simulink model "solution1_7009_CAN"  (R2017b)
settings: Solver=FixedStepAuto  StartTime=0.0  StopTime=inf  FixedStep=0.01  RelTol=1e-3
PostLoadFcn:
  | , if any(exist('dsrtsu_mdlpostloadfcn', 'file') == [2, 3, 6]), try dsrtsu_mdlpostloadfcn('Execute', bdroot); catch fprintf('Error in PostLoadFcn (dsrtsu_mdlpostloadfcn) for model "%s":\n %s\n', bdroot, lasterr); end, end,
values from neighbouring files (symbols this model uses):
  g = 9.81    [initialize_simplemodel.m]    (also in initialize_simplemodel_Trial.m; tire_friction_circle.m)
  h = 0.35    [initialize_simplemodel.m]    (also in initialize_simplemodel_Trial.m)
  lf = 1.4    [initialize_simplemodel.m]    (also in initialize_simplemodel_Trial.m)
  lr = 1.345    [initialize_simplemodel.m]    (also in initialize_simplemodel_Trial.m)
  m = 1400    [initialize_simplemodel.m]    (also in initialize_simplemodel_Trial.m = 1300; tire_friction_circle.m = 1300)
  r = 0.34    [initialize_simplemodel.m]    (also in initialize_simplemodel_Trial.m)
  tr = 1.684/2    (= 0.842)    [initialize_simplemodel.m]    (also in initialize_simplemodel_Trial.m)
  v_init = 60*5/18    (= 16.6666666667)    [initialize_simplemodel.m]    (also in initialize_simplemodel_Trial.m)
undefined symbols (not defined in the file or in its folder): DiscIntNeverNeededParam
libraries: simulink x27, rtican x10
(part 1 of 3)
settings Model: DSRTSU_INTERNAL_RTI_VER=510  DSRTSU_INTERNAL_RTI_TYPE=rti1401  Creator=ashwin.ramanujam  LastModifiedBy=Dell
settings DataIOCC: SignalLogging=off
settings HardwareCC: ProdBitPerPointer=32  ProdBitPerSizeT=32  ProdBitPerPtrDiffT=32  ProdLargestAtomicInteger=Integer  ProdEndianess=BigEndian  ProdWordSize=32  ProdHWDeviceType=Custom Processor->Custom  TargetIntDivRoundTo=Zero  TargetEndianess=BigEndian  TargetHWDeviceType=Custom Processor->Custom
settings SFSimCC: MATLABDynamicMemAlloc=off
settings RTWCC: SystemTargetFile=rti1401.tlc  MakeCommand=make_rti  TemplateMakefile=rti1401.tmf  Description=dSPACE DS1401 Hardware Platform
settings STFCustomTargetCC: ParMdlRefBuildCompliant=on  GRTInterface=off  SystemTargetFile=rti1401.tlc
settings GRTTargetCC: TargetLangStandard=C89/C90 (ANSI)  CompOptLevelCompliant=off  ConcurrentExecutionCompliant=off  CombineOutputUpdateFcns=off  MatFileLogging=off  CPPClassGenCompliant=off  UseToolchainInfoCompliant=off

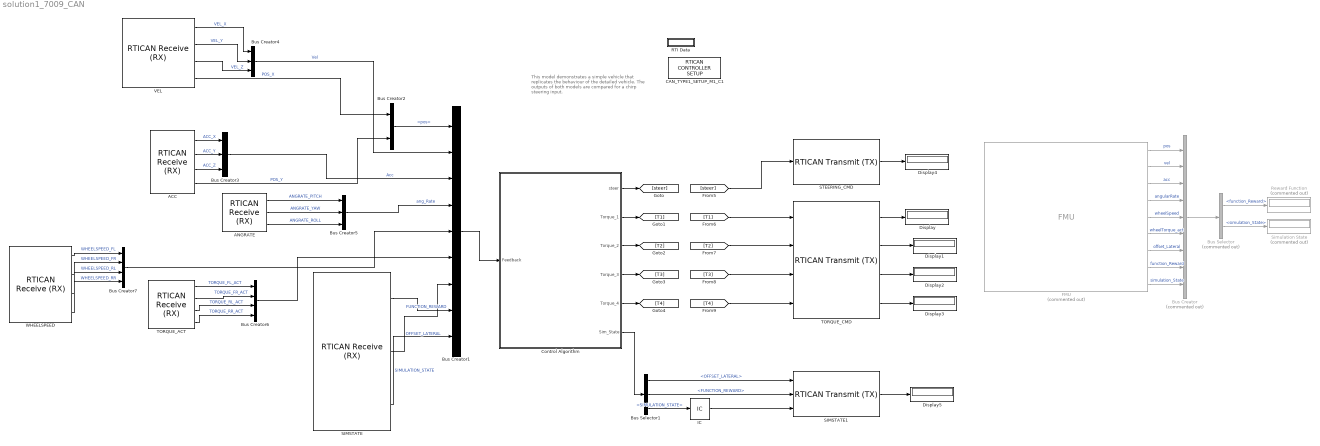
== system solution1_7009_CAN ==
  note: This model demonstrates a simple vehicle that replicates the behaviour of the detailed vehicle. The outputs of both models are compared for a chirp steering input.
  ACC : rtican/RTICAN Receive (RX)   Reserved1=[]  Reserved2=[]  Reserved3=[]  Reserved4=[]  SfcnMessage=[]  Msg_Struct=[]  BoardTypeNo=[]  BoardNo=[]  ChannelNo=[]  Parameters=[]  DialogFcn=[]  UnitName=[]  Revision=[]  UnitValues=[]  DSProperties=struct('RTI',struct('Version',uint32(5),'BlockType',struct('isSLSource',uint8(1),'isSLSink',uint8(1),'isHWSource',uint8(0),'isHWSink',uint8(0),'isSetup',uint8(0),'isInline',uint8(1),'isNonInline',uint8(0),'isInterrupt',uint8(0),'isChannelwise',uint8(0)),'IOBoardType','RTICAN','UnitType','MESSAGE','Identifier','RX','DialogType','MSVC','BlockSet','RTICAN','SlaveProcessor','CAN'))  RTIBlockInterface=struct('OutputPortsWidth',int32([1 1 1 1]),'OutputPortsActive',[1 1 1 1],'OutputPortsName',{{'ACC_X','ACC_Y','ACC_Z','POS_Y'}},'OutputPortsDataType',{{'SS_DOUBLE','SS_DOUBLE','SS_DOUBLE','SS_DOUBLE'}},'OutputPortsLabel',{{'ACC_X','ACC_Y','ACC_Z','POS_Y'}},'OutputPortsLabelMode','ON','InputPortsWidth',int32(0),'InputPortsActive',0,'DialogFcn','rtican_message_interface_gui','BlockDisplay',{{'','center'}},'IconTransparency','on','ParameterTunableNames',{{}},'InitLevel',3,'BlockName',struct('Token',{{'ACC'}}),'SampleTime',{{-1}},'TriggerPort',{{'none'}},'EnablePort',{{'none'}})  RTIBlockParameters=struct('BoardTypeNo',{{1,'OFF',[]}},'BoardNo',{{1,'ON',[1 16]}},'ChannelNo',{{1,'ON',[1 2]}},'Parameters',{{struct('DataFileSupport',struct('DataFileSelectedMaster',1,'DataFileSelectedLocal',1,'DataFileName','c:\users\dell\documents\github\rimac-stageb\challenge-resources\can-db\bus.dbc|','DataFileDate',{{{['02-Jun-2018 15:28:47']}}},'SelectedFile','..\..\challenge-resources\can-db\bus.dbc'),'Options',struct('StatusSelected',0,'TimeSelected',0,'DeltaTimeSelected',0,'BytePortSelected',0,'MessageLengthSelected',0,'TriggerPort',struct('Selected',0,'TriggerType',0),'UserCoding',struct('Selected',0,'InterfaceFile','UserDecodingFile','FcnName','UserDecodeFcn','InportSelected',0,'InportWidth',1,'OutportSelected',0,'OutportWidth',1),'EnablePortSelected',0,'SignalOnPortnameSelected',1,'UseRXService',0),'Message',struct('MsgOnBlocknameSelected',1,'MsgName','ACC','MsgIdFormat',0,'MsgId',4,'MsgLength',8,'NumSignals',4,'SampleTime',-1,'Signal',struct('SgnName',{'ACC_X','ACC_Y','ACC_Z','POS_Y'},'SgnStartBit',{0,16,32,48},'SgnLength',{16,16,16,16},'SgnType',{0,0,0,0},'ModeValue',{-1,-1,-1,-1},'DataType',{1,1,1,1},'ByteLayout',{0,0,0,0},'Factor',{0.0006,0.0006,0.0006,0.005},'Offset',{0,0,0,0},'SgnComment',{{''},{''},{''},{''}},'SgnUnit',{'m/s^2','m/s^2','m/s^2','m'},'Min',{-19.6608,-19.6608,-19.6608,-163.84},'Max',{19.6602,19.6602,19.6602,163.835},'SLDataType',{'SS_DOUBLE','SS_DOUBLE','SS_DOUBLE','SS_DOUBLE'}),'MsgIdNumFormat',0,'MsgComment',{{''}}),'Version',1.2,'general',struct('isFromLib',0)),'OFF',[]}},'GroupId',{{struct('Group',{{'RTICAN'}},'No',1,'Behavior',{{'NAMECHANGE'}},'BlockType',{{'SINK'}},'NameChangeFlag',0),'OFF',[]}},'SFcnRTICANMessage',{{struct('MsgType','RX','SFcnPortType','Scalar','MsgName','ACC','MsgIdFormat','STD','MsgId',4,'MsgLength',8,'NumSignals',4,'SampleTime',-1,'Signal',struct('SgnName',{'ACC_X','ACC_Y','ACC_Z','POS_Y'},'SgnStartBit',{0,16,32,48},'SgnLength',{16,16,16,16},'SgnType',{'standard','standard','standard','standard'},'ModeValue',{-1,-1,-1,-1},'DataType',{['signed int'],['signed int'],['signed int'],['signed int']},'ByteLayout',{['little endian'],['little endian'],['little endian'],['little endian']},'Factor',{0.0006,0.0006,0.0006,0.005},'Offset',{0,0,0,0},'SLDataType',{'SS_DOUBLE','SS_DOUBLE','SS_DOUBLE','SS_DOUBLE'}),'StatusSelected','no','TimeSelected','no','DeltaTimeSelected','no','BytePortSelected','no','MessageLengthSelected','no','TriggerPort',struct('Selected','no','TriggerType',0),'UserCoding',struct('Selected','no','InterfaceFile','UserDecodingFile','FcnName','UserDecodeFcn','InportSelected','no','InportWidth',1,'OutportSelected','no','OutportWidth',1),'EnablePortSelected','no','UseRXService','no','BoardType','DS1','BoardNo',1,'ControllerNo',1),'OFF',[]}},'TLCFileName',{{'rtican_rx_message','OFF',[]}})  RTISFcnParameters=struct('SFcnRTICANMessage','struct','TLCFileName','char')  RTIBlockParaDefault=struct('BoardTypeNo',4302,'BoardNo',1,'ChannelNo',1,'Parameters',struct('DataFileSupport',struct('DataFileSelectedMaster',0,'DataFileSelectedLocal',0,'DataFileName','','DataFileDate','','SelectedFile',['<no file selected>']),'Options',struct('StatusSelected',1,'TimeSelected',1,'DeltaTimeSelected',1,'BytePortSelected',0,'MessageLengthSelected',0,'TriggerPort',struct('Selected',0,'TriggerType','rising'),'UserCoding',struct('Selected',0,'InterfaceFile','UserDecodingFile','FcnName','UserDecodeFcn','InportSelected',0,'InportWidth',1,'OutportSelected',0,'OutportWidth',1),'EnablePortSelected',0,'SignalOnPortnameSelected',1,'UseRXService',0),'Message',struct('MsgOnBlocknameSelected',0,'MsgName',['RX Message'],'MsgIdFormat',0,'MsgId',100,'MsgLength',8,'NumSignals',1,'SampleTime',-1,'Signal',struct('SgnName',['RX signal'],'SgnStartBit',0,'SgnLength',8,'SgnType',0,'ModeValue',-1,'DataType',0,'SLDataType','SS_DOUBLE','ByteLayout',0,'Factor',1,'Offset',0,'Min',0,'Max',255,'SgnComment',{{}},'SgnUnit',''),'MsgIdNumFormat',0,'MsgComment',{{''}}),'Version',1.2,'general',struct('isFromLib',1)),'GroupId',struct('Group',{{'RTICAN'}},'No',1,'Behavior',{{'NAMECHANGE'}},'BlockType',{{'SINK'}},'NameChangeFlag',0),'SFcnRTICANMessage',struct('MsgType','RX','MsgName',['RX Message'],'MsgIdFormat','STD','MsgId',100,'MsgLength',8,'NumSignals',1,'SampleTime',-1,'Signal',struct('SgnName',['RX signal'],'SgnStartBit',0,'SgnLength',8,'SgnType','standard','ModeValue',-1,'DataType',['unsigned int'],'ByteLayout',['little endian'],'SLDataType','SS_DOUBLE','Factor',1,'Offset',0),'StatusSelected','yes','TimeSelected','yes','DeltaTimeSelected','yes','BytePortSelected','no','MessageLengthSelected','no','EnablePortSelected','no','UserCoding',struct('Selected','no','InterfaceFile','UserDecodingFile','FcnName','UserDecodeFcn','InportSelected','no','InportWidth',1,'OutportSelected','no','OutportWidth',1),'TriggerPort',struct('Selected','no','TriggerType','rising'),'UseRXService','no','BoardType','DS4302','BoardNo',1,'ControllerNo',1,'SFcnPortType','Scalar'),'TLCFileName','rtican_rx_message')
      settings: AttributesFormatString=Group Id: RTICAN1\n  SourceProductName=dSPACE RTI CAN Blockset
  ANGRATE : rtican/RTICAN Receive (RX)   Reserved1=[]  Reserved2=[]  Reserved3=[]  Reserved4=[]  SfcnMessage=[]  Msg_Struct=[]  BoardTypeNo=[]  BoardNo=[]  ChannelNo=[]  Parameters=[]  DialogFcn=[]  UnitName=[]  Revision=[]  UnitValues=[]  DSProperties=struct('RTI',struct('Version',uint32(5),'BlockType',struct('isSLSource',uint8(1),'isSLSink',uint8(1),'isHWSource',uint8(0),'isHWSink',uint8(0),'isSetup',uint8(0),'isInline',uint8(1),'isNonInline',uint8(0),'isInterrupt',uint8(0),'isChannelwise',uint8(0)),'IOBoardType','RTICAN','UnitType','MESSAGE','Identifier','RX','DialogType','MSVC','BlockSet','RTICAN','SlaveProcessor','CAN'))  RTIBlockInterface=struct('OutputPortsWidth',int32([1 1 1]),'OutputPortsActive',[1 1 1],'OutputPortsName',{{'ANGRATE_PITCH','ANGRATE_YAW','ANGRATE_ROLL'}},'OutputPortsDataType',{{'SS_DOUBLE','SS_DOUBLE','SS_DOUBLE'}},'OutputPortsLabel',{{'ANGRATE_PITCH','ANGRATE_YAW','ANGRATE_ROLL'}},'OutputPortsLabelMode','ON','InputPortsWidth',int32(0),'InputPortsActive',0,'DialogFcn','rtican_message_interface_gui','BlockDisplay',{{'','center'}},'IconTransparency','on','ParameterTunableNames',{{}},'InitLevel',3,'BlockName',struct('Token',{{'ANGRATE'}}),'SampleTime',{{-1}},'TriggerPort',{{'none'}},'EnablePort',{{'none'}})  RTIBlockParameters=struct('BoardTypeNo',{{1,'OFF',[]}},'BoardNo',{{1,'ON',[1 16]}},'ChannelNo',{{1,'ON',[1 2]}},'Parameters',{{struct('DataFileSupport',struct('DataFileSelectedMaster',1,'DataFileSelectedLocal',1,'DataFileName','c:\users\dell\documents\github\rimac-stageb\challenge-resources\can-db\bus.dbc|','DataFileDate',{{{['02-Jun-2018 15:28:47']}}},'SelectedFile','..\..\challenge-resources\can-db\bus.dbc'),'Options',struct('StatusSelected',0,'TimeSelected',0,'DeltaTimeSelected',0,'BytePortSelected',0,'MessageLengthSelected',0,'TriggerPort',struct('Selected',0,'TriggerType',0),'UserCoding',struct('Selected',0,'InterfaceFile','UserDecodingFile','FcnName','UserDecodeFcn','InportSelected',0,'InportWidth',1,'OutportSelected',0,'OutportWidth',1),'EnablePortSelected',0,'SignalOnPortnameSelected',1,'UseRXService',0),'Message',struct('MsgOnBlocknameSelected',1,'MsgName','ANGRATE','MsgIdFormat',0,'MsgId',5,'MsgLength',6,'NumSignals',3,'SampleTime',-1,'Signal',struct('SgnName',{'ANGRATE_PITCH','ANGRATE_YAW','ANGRATE_ROLL'},'SgnStartBit',{0,16,32},'SgnLength',{16,16,16},'SgnType',{0,0,0},'ModeValue',{-1,-1,-1},'DataType',{1,1,1},'ByteLayout',{0,0,0},'Factor',{0.001,0.001,0.001},'Offset',{0,0,0},'SgnComment',{{''},{''},{''}},'SgnUnit',{'rad/s','rad/s','rad/s'},'Min',{-32.768,-32.768,-32.768},'Max',{32.767,32.767,32.767},'SLDataType',{'SS_DOUBLE','SS_DOUBLE','SS_DOUBLE'}),'MsgIdNumFormat',0,'MsgComment',{{''}}),'Version',1.2,'general',struct('isFromLib',0)),'OFF',[]}},'GroupId',{{struct('Group',{{'RTICAN'}},'No',1,'Behavior',{{'NAMECHANGE'}},'BlockType',{{'SINK'}},'NameChangeFlag',0),'OFF',[]}},'SFcnRTICANMessage',{{struct('MsgType','RX','SFcnPortType','Scalar','MsgName','ANGRATE','MsgIdFormat','STD','MsgId',5,'MsgLength',6,'NumSignals',3,'SampleTime',-1,'Signal',struct('SgnName',{'ANGRATE_PITCH','ANGRATE_YAW','ANGRATE_ROLL'},'SgnStartBit',{0,16,32},'SgnLength',{16,16,16},'SgnType',{'standard','standard','standard'},'ModeValue',{-1,-1,-1},'DataType',{['signed int'],['signed int'],['signed int']},'ByteLayout',{['little endian'],['little endian'],['little endian']},'Factor',{0.001,0.001,0.001},'Offset',{0,0,0},'SLDataType',{'SS_DOUBLE','SS_DOUBLE','SS_DOUBLE'}),'StatusSelected','no','TimeSelected','no','DeltaTimeSelected','no','BytePortSelected','no','MessageLengthSelected','no','TriggerPort',struct('Selected','no','TriggerType',0),'UserCoding',struct('Selected','no','InterfaceFile','UserDecodingFile','FcnName','UserDecodeFcn','InportSelected','no','InportWidth',1,'OutportSelected','no','OutportWidth',1),'EnablePortSelected','no','UseRXService','no','BoardType','DS1','BoardNo',1,'ControllerNo',1),'OFF',[]}},'TLCFileName',{{'rtican_rx_message','OFF',[]}})  RTISFcnParameters=struct('SFcnRTICANMessage','struct','TLCFileName','char')  RTIBlockParaDefault=struct('BoardTypeNo',4302,'BoardNo',1,'ChannelNo',1,'Parameters',struct('DataFileSupport',struct('DataFileSelectedMaster',0,'DataFileSelectedLocal',0,'DataFileName','','DataFileDate','','SelectedFile',['<no file selected>']),'Options',struct('StatusSelected',1,'TimeSelected',1,'DeltaTimeSelected',1,'BytePortSelected',0,'MessageLengthSelected',0,'TriggerPort',struct('Selected',0,'TriggerType','rising'),'UserCoding',struct('Selected',0,'InterfaceFile','UserDecodingFile','FcnName','UserDecodeFcn','InportSelected',0,'InportWidth',1,'OutportSelected',0,'OutportWidth',1),'EnablePortSelected',0,'SignalOnPortnameSelected',1,'UseRXService',0),'Message',struct('MsgOnBlocknameSelected',0,'MsgName',['RX Message'],'MsgIdFormat',0,'MsgId',100,'MsgLength',8,'NumSignals',1,'SampleTime',-1,'Signal',struct('SgnName',['RX signal'],'SgnStartBit',0,'SgnLength',8,'SgnType',0,'ModeValue',-1,'DataType',0,'SLDataType','SS_DOUBLE','ByteLayout',0,'Factor',1,'Offset',0,'Min',0,'Max',255,'SgnComment',{{}},'SgnUnit',''),'MsgIdNumFormat',0,'MsgComment',{{''}}),'Version',1.2,'general',struct('isFromLib',1)),'GroupId',struct('Group',{{'RTICAN'}},'No',1,'Behavior',{{'NAMECHANGE'}},'BlockType',{{'SINK'}},'NameChangeFlag',0),'SFcnRTICANMessage',struct('MsgType','RX','MsgName',['RX Message'],'MsgIdFormat','STD','MsgId',100,'MsgLength',8,'NumSignals',1,'SampleTime',-1,'Signal',struct('SgnName',['RX signal'],'SgnStartBit',0,'SgnLength',8,'SgnType','standard','ModeValue',-1,'DataType',['unsigned int'],'ByteLayout',['little endian'],'SLDataType','SS_DOUBLE','Factor',1,'Offset',0),'StatusSelected','yes','TimeSelected','yes','DeltaTimeSelected','yes','BytePortSelected','no','MessageLengthSelected','no','EnablePortSelected','no','UserCoding',struct('Selected','no','InterfaceFile','UserDecodingFile','FcnName','UserDecodeFcn','InportSelected','no','InportWidth',1,'OutportSelected','no','OutportWidth',1),'TriggerPort',struct('Selected','no','TriggerType','rising'),'UseRXService','no','BoardType','DS4302','BoardNo',1,'ControllerNo',1,'SFcnPortType','Scalar'),'TLCFileName','rtican_rx_message')
      settings: AttributesFormatString=Group Id: RTICAN1\n  SourceProductName=dSPACE RTI CAN Blockset
  Bus Creator : BusCreator  Commented=on  Inputs=9
  Bus Creator1 : BusCreator  Inputs=9
  Bus Creator2 : BusCreator  Inputs=2
  Bus Creator3 : BusCreator  Inputs=3
  Bus Creator4 : BusCreator  Inputs=3
  Bus Creator5 : BusCreator  Inputs=3
  Bus Creator6 : BusCreator  Inputs=4
  Bus Creator7 : BusCreator  Inputs=4
  Bus Selector : BusSelector  Commented=on  OutputSignals=function_Reward,simulation_State
  Bus Selector1 : BusSelector  OutputSignals=OFFSET_LATERAL,FUNCTION_REWARD,SIMULATION_STATE
  CAN_TYPE1_SETUP_M1_C1 : rtican/RTICAN CONTROLLER SETUP   Reserved1=[]  Reserved2=[]  Reserved3=[]  Reserved4=[]  AcceptanceMask=[]  ArbitrationField=[]  Parameters=[]  SFcnRTICANSettings=[]  MS_Struct=[]  BoardTypeNo=[]  BoardNo=[]  ChannelNo=[]  DialogFcn=[]  UnitName=[]  Revision=[]  UnitValues=[]  DSProperties=struct('RTI',struct('Version',uint32(12),'BlockType',struct('isSLSource',uint8(0),'isSLSink',uint8(0),'isHWSource',uint8(0),'isHWSink',uint8(0),'isSetup',uint8(1),'isInline',uint8(1),'isNonInline',uint8(0),'isInterrupt',uint8(0),'isChannelwise',uint8(0)),'IOBoardType','RTICAN','UnitType','NON_MESSAGE','Identifier','MASTER','DialogType','ML','BlockSet','RTICAN','SlaveProcessor','CAN'))  RTIBlockInterface=struct('InputPortsWidth',int32(0),'InputPortsActive',0,'OutputPortsWidth',int32(0),'OutputPortsActive',0,'DialogFcn','rtican_master_setup_gui','BlockDisplay',{{['CAN CONTROLLER\n SETUP'],'center'}},'IconTransparency','on','InitLevel',3,'IWork',{{{'',uint32(2)}}},'BlockName',struct('Token',{{'CAN_TYPE','_SETUP_M','_C'}},'BlockParam',{{'BoardTypeNo','BoardNo','ChannelNo'}}),'ParameterTunableNames',{{}})  RTIBlockParameters="struct('BoardTypeNo',{{1,'OFF',[]}},'BoardNo',{{1,'ON',[1 16]}},'ChannelNo',{{1,'ON',[1 2]}},'AcceptanceMask',{{0,'OFF',[]}},'ArbitrationField',{{0,'OFF',[]}},'Parameters',{{struct('Config',struct('Baudrate',500,'SampleMode',1,'UsedParamSet',1,'validSettings',1,'isBTRvalues',0,'Advanced',struct('Baudrate',{500,500,500},'Frequency',{24000000,36000000,64000000},'Settings',{struct('SMPL',0,'BRP',0,'NBT',24,'TSEG1',15,'TSEG2',6,'SJW',3,'SP',70),struct('SMPL',0,'BRP',1,'NBT',18,'TSEG1',14,'TSEG2',1,'SJW',1,'SP',88),struct('SMPL',0,'BRP',3,'NBT',16,'TSEG1',12,'TSEG2',1,'SJW',1,'SP',87)},'BTR0',{192,65,67},'BTR1',{111,30,28})),'configType',1,'Options',struct('DataFileSelected',1,'DataFileName',{{'..\\..\\challenge-resources\\can-db\\bus.dbc'}},'DataFileDate',{{['02-Jun-2018 15:28:47']}},'InterfaceFcn','rtican_dbc_file_parser','InterfaceFcnFileName','','LabelConfigType','volatile','AcceptanceMaskSelected',0,'MsgDataType','AllwaysDouble','NumType','hex','MaskType','STD','AcceptanceMask',0,'ArbitrationField',0,'UseMultipleMessageAccess',0),'RxReceiveStdOptions',struct('RxServiceStdEnabled',0,'RxServiceStdMsgIdent',1000,'RxServiceStdIdentNumType',1,'RxServiceStdIdentMask',0,'RxServiceStdMaskNumType',1,'RxServiceStdQueueSize',64),'RxReceiveXtdOptions',struct('RxServiceXtdEnabled',0,'RxServiceXtdMsgIdent',1001,'RxServiceXtdIdentNumType',1,'RxServiceXtdIdentMask',0,'RxServiceXtdMaskNumType',1,'RxServiceXtdQueueSize',64),'PartialNetworkingOptions',struct('switchedon',0,'format',1,'idmask',['    XXXXX XXXXXXXX XXXXXXXX XXXXXXXX'],'idcode','0','idfilter','0','datamaskused',0,'datalength',1,'datamask','0x0000000000000000','partialnetworkenable',0),'general',struct('Termination_common',1,'Termination_C252',1,'BusConfigurationRegister',0,'Transceiver','ISO11898','isFromLib',0)),'OFF',[]}},'CCPParameters',{{struct('CRO',struct('Format','STD','NumFormat','hex','Id',1639),'DTO',struct('Format','STD','NumFormat','hex','Id',2017),'StationAdr',struct('NumFormat','hex','Value',57),'StationId',struct('Value',['dSPACE CCP Service']),'Enabled',0),'OFF',[]}},'XCPParameters',{{struct('MASTER',struct('Format','STD','NumFormat','hex','Id',256),'SLAVE',struct('Format','STD','NumFormat','hex','Id',510),'Enabled',0,'PIDTransmissionEnabled',0),'OFF',[]}},'GroupId',{{struct('Group',{{'RTICAN'}},'No',1,'Behavior',{{'EVER'}},'BlockType',{{'SOURCE'}},'NameChangeFlag',1),'OFF',[]}},'SFcnRTICANSettings',{{struct('Baudrate',500,'configType',1,'AdvancedConfig',struct('Frequency',{},'BTR0',{},'BTR1',{}),'UsedParamSet',1,'STDMaskSelected','no','XTDMaskSelected','no','BoardType','DS1','BoardNo',1,'ControllerNo',1,'Transceiver','ISO11898','BusConfigRegister',0,'TerminationRes',120,'UseMultipleMessageAccess','no','STDRXSrvcUsed','no','STDRXSrvcMsgId',1000,'STDRXSrvcMsgMask',0,'STDRXSrvcQueueSize',64,'XTDRXSrvcUsed','no','XTDRXSrvcMsgId',1001,'XTDRXSrvcQueueSize',64,'XTDRXSrvcMsgMask',0,'PN_IsPNTransciever',0,'PN_IsPNEnabled',0,'PN_MsgFormat',1,'PN_idcode',0,'PN_idmask',2047,'PN_datamaskused',0,'PN_datalength',0,'PN_datamask',['0xFF, 0xFF, 0xFF, 0xFF, 0xFF, 0xFF, 0xFF, 0xFF']),'OFF',[]}},'SFcnRTICCPSettings',{{struct('CRO',struct('Format','STD','NumFormat','hex','Id',1639),'DTO',struct('Format','STD','NumFormat','hex','Id',2017),'StationAdr',struct('NumFormat','hex','Value',57),'StationId',struct('Value',['dSPACE CCP Service']),'Enabled',0),'OFF',[]}},'SFcnRTIXCPSettings',{{struct('MASTER',struct('Format','STD','NumFormat','hex','Id',256),'SLAVE',struct('Format','STD','NumFormat','hex','Id',510),'Enabled',0,'PIDTransmissionEnabled',0),'OFF',[]}},'TLCFileName',{{'rtican_master_setup','OFF',[]}})"  RTISFcnParameters=struct('SFcnRTICANSettings','struct','SFcnRTICCPSettings','struct','SFcnRTIXCPSettings','struct','AcceptanceMask','int32','ArbitrationField','int32','TLCFileName','char')  RTIBlockParaDefault="struct('BoardTypeNo',4302,'BoardNo',1,'ChannelNo',1,'AcceptanceMask',0,'ArbitrationField',0,'Parameters',struct('Config',struct('Baudrate',500,'SampleMode',1,'UsedParamSet',1,'validSettings',1,'isBTRvalues',0,'Advanced',struct('Frequency',16000000,'BTR0',64,'BTR1',28,'Settings',struct('SMPL',0,'BRP',0,'NBT',16,'TSEG1',12,'TSEG2',1,'SJW',1,'SP',87))),'configType',1,'Options',struct('DataFileSelected',0,'DataFileName',{{['<no datafile support>']}},'DataFileDate',{{''}},'InterfaceFcn','rtican_dbc_file_parser','InterfaceFcnFileName','','LabelConfigType','volatile','AcceptanceMaskSelected',0,'MsgDataType','AllwaysDouble','NumType','hex','MaskType','STD','AcceptanceMask',0,'ArbitrationField',0,'UseMultipleMessageAccess',0),'RxReceiveStdOptions',struct('RxServiceStdEnabled',0,'RxServiceStdMsgIdent',1000,'RxServiceStdIdentNumType',1,'RxServiceStdIdentMask',0,'RxServiceStdMaskNumType',1,'RxServiceStdQueueSize',64),'RxReceiveXtdOptions',struct('RxServiceXtdEnabled',0,'RxServiceXtdMsgIdent',1001,'RxServiceXtdIdentNumType',1,'RxServiceXtdIdentMask',0,'RxServiceXtdMaskNumType',1,'RxServiceXtdQueueSize',64),'PartialNetworkingOptions',struct('switchedon',0,'format',1,'idmask',['    XXXXX XXXXXXXX XXXXXXXX XXXXXXXX'],'idcode','0','idfilter','0','datamaskused',0,'datalength',1,'datamask','0x0000000000000000','partialnetworkenable',0),'general',struct('Termination_common',1,'Termination_C252',1,'BusConfigurationRegister',0,'Transceiver','ISO11898','isFromLib',1)),'CCPParameters',struct('CRO',struct('Format','STD','NumFormat','hex','Id',1639),'DTO',struct('Format','STD','NumFormat','hex','Id',2017),'StationAdr',struct('NumFormat','hex','Value',57),'StationId',struct('Value',['dSPACE CCP Service']),'Enabled',0),'XCPParameters',struct('MASTER',struct('Format','STD','NumFormat','hex','Id',256),'SLAVE',struct('Format','STD','NumFormat','hex','Id',510),'Enabled',0,'PIDTransmissionEnabled',0),'GroupId',struct('Group',{{'RTICAN'}},'No',1,'Behavior',{{'EVER'}},'BlockType',{{'SOURCE'}},'NameChangeFlag',1),'SFcnRTICANSettings',struct('Baudrate',500,'configType',1,'AdvandedConfig',struct('Frequency',16000000,'BTR0','0x40','BTR1','0x1C'),'UsedParamSet',1,'STDMaskSelected','no','XTDMaskSelected','no','BoardType','DS4302','BoardNo',1,'ControllerNo',1,'Transceiver','ISO11898','BusConfigRegister',0,'TerminationRes',120,'UseMultipleMessageAccess','no','STDRXSrvcUsed','no','STDRXSrvcMsgId',1000,'STDRXSrvcMsgMask',0,'STDRXSrvcQueueSize',64,'XTDRXSrvcUsed','no','XTDRXSrvcMsgId',1001,'XTDRXSrvcQueueSize',64,'XTDRXSrvcMsgMask',0),'SFcnRTICCPSettings',struct('CRO',struct('Format','STD','NumFormat','hex','Id',1639),'DTO',struct('Format','STD','NumFormat','hex','Id',2017),'StationAdr',struct('NumFormat','hex','Value',57),'StationId',struct('Value',['dSPACE CCP Service']),'Enabled',0),'SFcnRTIXCPSettings',struct('MASTER',struct('Format','STD','NumFormat','hex','Id',256),'SLAVE',struct('Format','STD','NumFormat','hex','Id',510),'Enabled',0,'PIDTransmissionEnabled',0),'TLCFileName','rtican_master_setup')"
      settings: AttributesFormatString=Group Id: RTICAN1\n  SourceProductName=dSPACE RTI CAN Blockset
  Control Algorithm : Subsystem
  Display{,1..5} (6 alike) : Display
  FMU : FMU  Commented=on  FMUName=MED2018_VehicleModel.fmu  FMUMode=CoSimulation  FMUSampleTime=-1  mask(MED2018.VehicleModel [Co-Simulation, v2.0]){}
      mask Display:
      | if (exist([Simulink.fileGenControl('get','CacheFolder') '\slprj\_fmu\9cdf7761f2cda4d0241d3dfb8ea8a77c\MED2018_VehicleModel\model.png'],'file'))
      |     image([Simulink.fileGenControl('get','CacheFolder') '\slprj\_fmu\9cdf7761f2cda4d0241d3dfb8ea8a77c\MED2018_VehicleModel\model.png']);
      |     text(0.03, 0.97, 'MED2018.VehicleModel', 'horizontalAlignment', 'left', 'verticalAlignment', 'top');
      | else
      |     disp('MED2018.VehicleModel');
      | end
      | port_label('output',1,'Position');
      | port_label('output',2,'Velocity');
      | port_label('output',3,'Acceleration');
      | port_label('output',4,'angularRate');
      | port_label('output',5,'wheelSpeed');
      | port_label('output',6,'wheelTorque_act');
      | port_label('output',7,'offset_Lateral');
      | port_label('output',8,'function_Reward');
      | port_label('output',9,'simulation_State');
      | port_label('input',1,'steering_Angle');
      | port_label('input',2,'wheelTorque_cmd_FL');
      | port_label('input',3,'wheelTorque_cmd_FR');
      | port_label('input',4,'wheelTorque_cmd_RL');
      | port_label('input',5,'wheelTorque_cmd_RR');
  IC : InitialCondition
  RTI Data : Subsystem  Tag=struct('RTIDataServer',struct('RTIDataServerVs','2','RTIModelDescription','struct(''main'',''solution1_7009_CAN'',''sub'','''',''isMp'',0)'))  LoadFcn="if exist('rtidc'), try,  rtidc('DataHostBlockClbLoad', gcbh); catch, disp(['Warning: ''LoadFcn'' for RTI Data block failed: ' lasterr]); end, end,"  mask(RTI_DATA_HOST){}
      mask help:
      | RTI Data Block.
      | This block is used by RTI to store internal model-dependent data.
      | Please keep this block on the root level of the model. Deleting this block will result in data loss.
      |
      | NEVER DELETE OR COPY THIS BLOCK!
      settings: CopyFcn="if exist('rtidc'), try,  rtidc('DataHostBlockClbCopy', gcbh); catch, disp(['Warning: ''CopyFcn'' for RTI Data block failed: ' lasterr]); end, end,"  DeleteFcn="if exist('rtidc'), try,  rtidc('DataHostBlockClbDelete', gcbh); catch, disp(['Warning: ''DeleteFcn'' for RTI Data block failed: ' lasterr]); end, end,"  ModelCloseFcn="if exist('rtidc'), try,  rtidc('DataHostBlockClbModelClose', gcbh); catch, disp(['Warning: ''ModelCloseFcn'' for RTI Data block failed: ' lasterr]); end, end,"  PreSaveFcn="if exist('rtidc'), try,  rtidc('DataHostBlockClbPreSave', gcbh); catch, disp(['Warning: ''PreSaveFcn'' for RTI Data block failed: ' lasterr]); end, end,"  PostSaveFcn="if exist('rtidc'), try,  rtidc('DataHostBlockClbPostSave', gcbh); catch, disp(['Warning: ''PostSaveFcn'' for RTI Data block failed: ' lasterr]); end, end,"  NameChangeFcn="if exist('rtidc'), try,  rtidc('DataHostBlockClbNameChange', gcbh); catch, disp(['Warning: ''NameChangeFcn'' for RTI Data block failed: ' lasterr]); end, end,"
      mask Help:
      | RTI Data Block.
      | This block is used by RTI to store internal model-dependent data.
      | Please keep this block on the root level of the model. Deleting this block will result in data loss.
      | 
      | NEVER DELETE OR COPY THIS BLOCK!
      mask Display:
      | text(0.5, 0.5, 'RTI Data', 'HorizontalAlignment', 'center');
      | plot([1 0]);
  Reward Function : Display  Commented=on
  SIMSTATE : rtican/RTICAN Receive (RX)   Reserved1=[]  Reserved2=[]  Reserved3=[]  Reserved4=[]  SfcnMessage=[]  Msg_Struct=[]  BoardTypeNo=[]  BoardNo=[]  ChannelNo=[]  Parameters=[]  DialogFcn=[]  UnitName=[]  Revision=[]  UnitValues=[]  DSProperties=struct('RTI',struct('Version',uint32(5),'BlockType',struct('isSLSource',uint8(1),'isSLSink',uint8(1),'isHWSource',uint8(0),'isHWSink',uint8(0),'isSetup',uint8(0),'isInline',uint8(1),'isNonInline',uint8(0),'isInterrupt',uint8(0),'isChannelwise',uint8(0)),'IOBoardType','RTICAN','UnitType','MESSAGE','Identifier','RX','DialogType','MSVC','BlockSet','RTICAN','SlaveProcessor','CAN'))  RTIBlockInterface=struct('OutputPortsWidth',int32([1 1 1]),'OutputPortsActive',[1 1 1],'OutputPortsName',{{'FUNCTION_REWARD','OFFSET_LATERAL','SIMULATION_STATE'}},'OutputPortsDataType',{{'SS_DOUBLE','SS_DOUBLE','SS_DOUBLE'}},'OutputPortsLabel',{{'FUNCTION_REWARD','OFFSET_LATERAL','SIMULATION_STATE'}},'OutputPortsLabelMode','ON','InputPortsWidth',int32(0),'InputPortsActive',0,'DialogFcn','rtican_message_interface_gui','BlockDisplay',{{'','center'}},'IconTransparency','on','ParameterTunableNames',{{}},'InitLevel',3,'BlockName',struct('Token',{{'SIMSTATE'}}),'SampleTime',{{-1}},'TriggerPort',{{'none'}},'EnablePort',{{'none'}})  RTIBlockParameters=struct('BoardTypeNo',{{1,'OFF',[]}},'BoardNo',{{1,'ON',[1 16]}},'ChannelNo',{{1,'ON',[1 2]}},'Parameters',{{struct('DataFileSupport',struct('DataFileSelectedMaster',1,'DataFileSelectedLocal',1,'DataFileName','c:\users\dell\documents\github\rimac-stageb\challenge-resources\can-db\bus.dbc|','DataFileDate',{{{['02-Jun-2018 15:28:47']}}},'SelectedFile','..\..\challenge-resources\can-db\bus.dbc'),'Options',struct('StatusSelected',0,'TimeSelected',0,'DeltaTimeSelected',0,'BytePortSelected',0,'MessageLengthSelected',0,'TriggerPort',struct('Selected',0,'TriggerType',0),'UserCoding',struct('Selected',0,'InterfaceFile','UserDecodingFile','FcnName','UserDecodeFcn','InportSelected',0,'InportWidth',1,'OutportSelected',0,'OutportWidth',1),'EnablePortSelected',0,'SignalOnPortnameSelected',1,'UseRXService',0),'Message',struct('MsgOnBlocknameSelected',1,'MsgName','SIMSTATE','MsgIdFormat',0,'MsgId',8,'MsgLength',5,'NumSignals',3,'SampleTime',-1,'Signal',struct('SgnName',{'FUNCTION_REWARD','OFFSET_LATERAL','SIMULATION_STATE'},'SgnStartBit',{0,16,24},'SgnLength',{16,8,2},'SgnType',{0,0,0},'ModeValue',{-1,-1,-1},'DataType',{0,1,1},'ByteLayout',{0,0,0},'Factor',{0.015,0.05,1},'Offset',{0,0,0},'SgnComment',{{''},{''},{''}},'SgnUnit',{'','m',''},'Min',{0,-6.4,0},'Max',{983.025,6.35,4},'SLDataType',{'SS_DOUBLE','SS_DOUBLE','SS_DOUBLE'}),'MsgIdNumFormat',0,'MsgComment',{{''}}),'Version',1.2,'general',struct('isFromLib',0)),'OFF',[]}},'GroupId',{{struct('Group',{{'RTICAN'}},'No',1,'Behavior',{{'NAMECHANGE'}},'BlockType',{{'SINK'}},'NameChangeFlag',0),'OFF',[]}},'SFcnRTICANMessage',{{struct('MsgType','RX','SFcnPortType','Scalar','MsgName','SIMSTATE','MsgIdFormat','STD','MsgId',8,'MsgLength',5,'NumSignals',3,'SampleTime',-1,'Signal',struct('SgnName',{'FUNCTION_REWARD','OFFSET_LATERAL','SIMULATION_STATE'},'SgnStartBit',{0,16,24},'SgnLength',{16,8,2},'SgnType',{'standard','standard','standard'},'ModeValue',{-1,-1,-1},'DataType',{['unsigned int'],['signed int'],['signed int']},'ByteLayout',{['little endian'],['little endian'],['little endian']},'Factor',{0.015,0.05,1},'Offset',{0,0,0},'SLDataType',{'SS_DOUBLE','SS_DOUBLE','SS_DOUBLE'}),'StatusSelected','no','TimeSelected','no','DeltaTimeSelected','no','BytePortSelected','no','MessageLengthSelected','no','TriggerPort',struct('Selected','no','TriggerType',0),'UserCoding',struct('Selected','no','InterfaceFile','UserDecodingFile','FcnName','UserDecodeFcn','InportSelected','no','InportWidth',1,'OutportSelected','no','OutportWidth',1),'EnablePortSelected','no','UseRXService','no','BoardType','DS1','BoardNo',1,'ControllerNo',1),'OFF',[]}},'TLCFileName',{{'rtican_rx_message','OFF',[]}})  RTISFcnParameters=struct('SFcnRTICANMessage','struct','TLCFileName','char')  RTIBlockParaDefault=struct('BoardTypeNo',4302,'BoardNo',1,'ChannelNo',1,'Parameters',struct('DataFileSupport',struct('DataFileSelectedMaster',0,'DataFileSelectedLocal',0,'DataFileName','','DataFileDate','','SelectedFile',['<no file selected>']),'Options',struct('StatusSelected',1,'TimeSelected',1,'DeltaTimeSelected',1,'BytePortSelected',0,'MessageLengthSelected',0,'TriggerPort',struct('Selected',0,'TriggerType','rising'),'UserCoding',struct('Selected',0,'InterfaceFile','UserDecodingFile','FcnName','UserDecodeFcn','InportSelected',0,'InportWidth',1,'OutportSelected',0,'OutportWidth',1),'EnablePortSelected',0,'SignalOnPortnameSelected',1,'UseRXService',0),'Message',struct('MsgOnBlocknameSelected',0,'MsgName',['RX Message'],'MsgIdFormat',0,'MsgId',100,'MsgLength',8,'NumSignals',1,'SampleTime',-1,'Signal',struct('SgnName',['RX signal'],'SgnStartBit',0,'SgnLength',8,'SgnType',0,'ModeValue',-1,'DataType',0,'SLDataType','SS_DOUBLE','ByteLayout',0,'Factor',1,'Offset',0,'Min',0,'Max',255,'SgnComment',{{}},'SgnUnit',''),'MsgIdNumFormat',0,'MsgComment',{{''}}),'Version',1.2,'general',struct('isFromLib',1)),'GroupId',struct('Group',{{'RTICAN'}},'No',1,'Behavior',{{'NAMECHANGE'}},'BlockType',{{'SINK'}},'NameChangeFlag',0),'SFcnRTICANMessage',struct('MsgType','RX','MsgName',['RX Message'],'MsgIdFormat','STD','MsgId',100,'MsgLength',8,'NumSignals',1,'SampleTime',-1,'Signal',struct('SgnName',['RX signal'],'SgnStartBit',0,'SgnLength',8,'SgnType','standard','ModeValue',-1,'DataType',['unsigned int'],'ByteLayout',['little endian'],'SLDataType','SS_DOUBLE','Factor',1,'Offset',0),'StatusSelected','yes','TimeSelected','yes','DeltaTimeSelected','yes','BytePortSelected','no','MessageLengthSelected','no','EnablePortSelected','no','UserCoding',struct('Selected','no','InterfaceFile','UserDecodingFile','FcnName','UserDecodeFcn','InportSelected','no','InportWidth',1,'OutportSelected','no','OutportWidth',1),'TriggerPort',struct('Selected','no','TriggerType','rising'),'UseRXService','no','BoardType','DS4302','BoardNo',1,'ControllerNo',1,'SFcnPortType','Scalar'),'TLCFileName','rtican_rx_message')
      settings: AttributesFormatString=Group Id: RTICAN1\n  SourceProductName=dSPACE RTI CAN Blockset
  SIMSTATE1 : rtican/RTICAN Transmit (TX)   Reserved1=[]  Reserved2=[]  Reserved3=[]  Reserved4=[]  SfcnMessage=[]  Msg_Struct=[]  BoardTypeNo=[]  BoardNo=[]  ChannelNo=[]  Parameters=[]  DialogFcn=[]  UnitName=[]  Revision=[]  UnitValues=[]  DSProperties=struct('RTI',struct('Version',uint32(5),'BlockType',struct('isSLSource',uint8(1),'isSLSink',uint8(1),'isHWSource',uint8(0),'isHWSink',uint8(0),'isSetup',uint8(0),'isInline',uint8(1),'isNonInline',uint8(0),'isInterrupt',uint8(0),'isChannelwise',uint8(0)),'IOBoardType','RTICAN','UnitType','MESSAGE','Identifier','TX','DialogType','MSVC','BlockSet','RTICAN','SlaveProcessor','CAN'))  RTIBlockInterface=struct('InputPortsWidth',int32([1 1 1]),'InputPortsActive',[1 1 1],'InputPortsName',{{'FUNCTION_REWARD','OFFSET_LATERAL','SIMULATION_STATE'}},'InputPortsDataType',{{'SS_DOUBLE','SS_DOUBLE','SS_DOUBLE'}},'OutputPortsWidth',int32(1),'OutputPortsActive',1,'OutputPortsName',{{['TX delay time']}},'DialogFcn','rtican_message_interface_gui','BlockDisplay',{{'','center'}},'IconTransparency','on','InitLevel',3,'BlockName',struct('Token',{{'SIMSTATE'}}),'SampleTime',{{-1}},'TriggerPort',{{'none'}},'EnablePort',{{'none'}})  RTIBlockParameters=struct('BoardTypeNo',{{1,'OFF',[]}},'BoardNo',{{1,'ON',[1 16]}},'ChannelNo',{{1,'ON',[1 2]}},'Parameters',{{struct('DataFileSupport',struct('DataFileSelectedMaster',1,'DataFileSelectedLocal',1,'DataFileName','c:\users\dell\documents\github\rimac-stageb\challenge-resources\can-db\bus.dbc|','DataFileDate',{{{['02-Jun-2018 15:28:47']}}},'SelectedFile','..\..\challenge-resources\can-db\bus.dbc'),'Options',struct('StatusSelected',0,'TimeSelected',0,'DeltaTimeSelected',0,'DelayTimeSelected',1,'DelayTimeTXCommandSelected',0,'EncodeSetUnusedBitsToOne',0,'EnableMsgLoopback',0,'TriggerPort',struct('Selected',0,'TriggerType',0),'EnablePortSelected',0,'SignalOnPortnameSelected',1,'UserCoding',struct('Selected',0,'InterfaceFile','UserEncodingFile','FcnName','UserEncodeFcn','InportSelected',0,'InportWidth',1,'OutportSelected',0,'OutportWidth',1),'TerminationMsg',struct('Selected',0,'Byte0_7','0'),'InitialMsg',struct('Selected',0,'Byte0_7','0')),'Message',struct('MsgOnBlocknameSelected',1,'MsgName','SIMSTATE','MsgIdFormat',0,'MsgId',8,'MsgLength',5,'NumSignals',3,'SampleTime',-1,'StartTime',struct('Selected',0,'Value',0),'AutoRepeatTime',struct('Selected',0,'Value',0.1),'Timeout',struct('Selected',0,'Value',0.1),'DelayTime',struct('Selected',0,'Value',0.1),'Signal',struct('SgnName',{'FUNCTION_REWARD','OFFSET_LATERAL','SIMULATION_STATE'},'SgnStartBit',{0,16,24},'SgnLength',{16,8,2},'SgnType',{0,0,0},'ModeValue',{-1,-1,-1},'DataType',{0,1,1},'ByteLayout',{0,0,0},'Factor',{0.015,0.05,1},'Offset',{0,0,0},'SgnComment',{{''},{''},{''}},'SgnUnit',{'','m',''},'Min',{0,-6.4,0},'Max',{983.025,6.35,4},'SLDataType',{'SS_DOUBLE','SS_DOUBLE','SS_DOUBLE'}),'MsgIdNumFormat',0,'MsgComment',{{''}}),'Version',1.2,'general',struct('isFromLib',0)),'OFF',[]}},'GroupId',{{struct('Group',{{'RTICAN'}},'No',1,'Behavior',{{'NAMECHANGE'}},'BlockType',{{'SINK'}},'NameChangeFlag',0),'OFF',[]}},'SFcnRTICANMessage',{{struct('MsgType','TX','SFcnPortType','Scalar','MsgName','SIMSTATE','MsgIdFormat','STD','MsgId',8,'MsgLength',5,'NumSignals',3,'SampleTime',-1,'StartTime',struct('Selected','no','Value',0),'AutoRepeatTime',struct('Selected','no','Value',0.1),'Timeout',struct('Selected','no','Value',0.1),'Signal',struct('SgnName',{'FUNCTION_REWARD','OFFSET_LATERAL','SIMULATION_STATE'},'SgnStartBit',{0,16,24},'SgnLength',{16,8,2},'SgnType',{'standard','standard','standard'},'ModeValue',{-1,-1,-1},'DataType',{['unsigned int'],['signed int'],['signed int']},'ByteLayout',{['little endian'],['little endian'],['little endian']},'Factor',{0.015,0.05,1},'Offset',{0,0,0},'SLDataType',{'SS_DOUBLE','SS_DOUBLE','SS_DOUBLE'}),'StatusSelected','no','TimeSelected','no','DeltaTimeSelected','no','DelayTimeSelected','yes','DelayTimeTXCommandSelected','no','EncodeSetUnusedBitsToOne','no','EnableMsgLoopback','no','TriggerPort',struct('Selected','no','TriggerType',0),'EnablePortSelected','no','UserCoding',struct('Selected','no','InterfaceFile','UserEncodingFile','FcnName','UserEncodeFcn','InportSelected','no','InportWidth',1,'OutportSelected','no','OutportWidth',1),'TerminationMsg',struct('Selected','no','Byte0','0x00','Byte1','0x00','Byte2','0x00','Byte3','0x00','Byte4','0x00','Byte5','0x00','Byte6','0x00','Byte7','0x00'),'InitialMsg',struct('Selected','no','Byte0','0x00','Byte1','0x00','Byte2','0x00','Byte3','0x00','Byte4','0x00','Byte5','0x00','Byte6','0x00','Byte7','0x00'),'BoardType','DS1','BoardNo',1,'ControllerNo',1),'OFF',[]}},'TLCFileName',{{'rtican_tx_message','OFF',[]}})  RTISFcnParameters=struct('SFcnRTICANMessage','struct','TLCFileName','char')  RTIBlockParaDefault=struct('BoardTypeNo',4302,'BoardNo',1,'ChannelNo',1,'Parameters',struct('DataFileSupport',struct('DataFileSelectedMaster',0,'DataFileSelectedLocal',0,'DataFileName','','DataFileDate','','SelectedFile',['<no file selected>']),'Options',struct('StatusSelected',1,'TimeSelected',1,'DeltaTimeSelected',1,'DelayTimeSelected',1,'DelayTimeTXCommandSelected',0,'EncodeSetUnusedBitsToOne',0,'EnableMsgLoopback',0,'TriggerPort',struct('Selected',0,'TriggerType','rising'),'EnablePortSelected',0,'SignalOnPortnameSelected',1,'UserCoding',struct('Selected',0,'InterfaceFile','UserEncodingFile','FcnName','UserEncodeFcn','InportSelected',0,'InportWidth',1,'OutportSelected',0,'OutportWidth',1),'TerminationMsg',struct('Selected',0,'Byte0_7','0'),'InitialMsg',struct('Selected',0,'Byte0_7','0')),'Message',struct('MsgOnBlocknameSelected',0,'MsgName',['TX Message'],'MsgIdFormat',0,'MsgId',100,'MsgLength',8,'NumSignals',1,'SampleTime',-1,'StartTime',struct('Selected',0,'Value',0),'AutoRepeatTime',struct('Selected',0,'Value',0.1),'Timeout',struct('Selected',0,'Value',0.1),'DelayTime',struct('Selected',0,'Value',0.1),'Signal',struct('SgnName',['TX signal'],'SgnStartBit',0,'SgnLength',8,'SgnType',0,'ModeValue',-1,'DataType',0,'SLDataType','SS_DOUBLE','ByteLayout',0,'Factor',1,'Offset',0,'Min',0,'Max',255,'SgnComment',{{}},'SgnUnit',''),'MsgIdNumFormat',0,'MsgComment',{{''}}),'Version',1.2,'general',struct('isFromLib',1)),'GroupId',struct('Group',{{'RTICAN'}},'No',1,'Behavior',{{'NAMECHANGE'}},'BlockType',{{'SINK'}},'NameChangeFlag',0),'SFcnRTICANMessage',struct('MsgType','TX','MsgName',['TX Message'],'MsgIdFormat','STD','MsgId',100,'MsgLength',2,'NumSignals',1,'SampleTime',-1,'StartTime',struct('Selected','no','Value',0),'AutoRepeatTime',struct('Selected','no','Value',0.1),'Timeout',struct('Selected','no','Value',0.1),'DelayTime',struct('Selected','no','Value',0.1),'Signal',struct('SgnName',['TX signal'],'SgnStartBit',0,'SgnLength',8,'SgnType','standard','ModeValue',-1,'DataType',['unsigned int'],'ByteLayout',['little endian'],'SLDataType','SS_DOUBLE','Factor',1,'Offset',0),'StatusSelected','yes','TimeSelected','yes','DeltaTimeSelected','yes','DelayTimeSelected','yes','EnablePortSelected','no','EnableMsgLoopback','no','DelayTimeTXCommandSelected','no','EncodeSetUnusedBitsToOne','no','UserCoding',struct('Selected','no','InterfaceFile','UserDecodingFile','FcnName','UserDecodeFcn','InportSelected','no','InportWidth',1,'OutportSelected','no','OutportWidth',1),'TerminationMsg',struct('Selected','no','Byte0','0x00','Byte1','0x00','Byte2','0x00','Byte3','0x00','Byte4','0x00','Byte5','0x00','Byte6','0x00','Byte7','0x00'),'InitialMsg',struct('Selected','no','Byte0','0x00','Byte1','0x00','Byte2','0x00','Byte3','0x00','Byte4','0x00','Byte5','0x00','Byte6','0x00','Byte7','0x00'),'TriggerPort',struct('Selected','no','TriggerType','rising'),'BoardType','DS4302','BoardNo',1,'ControllerNo',1,'SFcnPortType','Scalar'),'TLCFileName','rtican_tx_message')
      settings: AttributesFormatString=Group Id: RTICAN1\n  SourceProductName=dSPACE RTI CAN Blockset
  STEERING_CMD : rtican/RTICAN Transmit (TX)   Reserved1=[]  Reserved2=[]  Reserved3=[]  Reserved4=[]  SfcnMessage=[]  Msg_Struct=[]  BoardTypeNo=[]  BoardNo=[]  ChannelNo=[]  Parameters=[]  DialogFcn=[]  UnitName=[]  Revision=[]  UnitValues=[]  DSProperties=struct('RTI',struct('Version',uint32(5),'BlockType',struct('isSLSource',uint8(1),'isSLSink',uint8(1),'isHWSource',uint8(0),'isHWSink',uint8(0),'isSetup',uint8(0),'isInline',uint8(1),'isNonInline',uint8(0),'isInterrupt',uint8(0),'isChannelwise',uint8(0)),'IOBoardType','RTICAN','UnitType','MESSAGE','Identifier','TX','DialogType','MSVC','BlockSet','RTICAN','SlaveProcessor','CAN'))  RTIBlockInterface=struct('InputPortsWidth',int32(1),'InputPortsActive',1,'InputPortsName',{{'STEERING_ANGLE_CMD'}},'InputPortsDataType',{{'SS_DOUBLE'}},'OutputPortsWidth',int32(1),'OutputPortsActive',1,'OutputPortsName',{{['TX delay time']}},'DialogFcn','rtican_message_interface_gui','BlockDisplay',{{'','center'}},'IconTransparency','on','InitLevel',3,'BlockName',struct('Token',{{'STEERING_CMD'}}),'SampleTime',{{-1}},'TriggerPort',{{'none'}},'EnablePort',{{'none'}})  RTIBlockParameters=struct('BoardTypeNo',{{1,'OFF',[]}},'BoardNo',{{1,'ON',[1 16]}},'ChannelNo',{{1,'ON',[1 2]}},'Parameters',{{struct('DataFileSupport',struct('DataFileSelectedMaster',1,'DataFileSelectedLocal',1,'DataFileName','c:\users\dell\documents\github\rimac-stageb\challenge-resources\can-db\bus.dbc|','DataFileDate',{{{['02-Jun-2018 15:28:47']}}},'SelectedFile','..\..\challenge-resources\can-db\bus.dbc'),'Options',struct('StatusSelected',0,'TimeSelected',0,'DeltaTimeSelected',0,'DelayTimeSelected',1,'DelayTimeTXCommandSelected',0,'EncodeSetUnusedBitsToOne',0,'EnableMsgLoopback',0,'TriggerPort',struct('Selected',0,'TriggerType',0),'EnablePortSelected',0,'SignalOnPortnameSelected',1,'UserCoding',struct('Selected',0,'InterfaceFile','UserEncodingFile','FcnName','UserEncodeFcn','InportSelected',0,'InportWidth',1,'OutportSelected',0,'OutportWidth',1),'TerminationMsg',struct('Selected',0,'Byte0_7','0'),'InitialMsg',struct('Selected',0,'Byte0_7','0')),'Message',struct('MsgOnBlocknameSelected',1,'MsgName','STEERING_CMD','MsgIdFormat',0,'MsgId',1,'MsgLength',2,'NumSignals',1,'SampleTime',-1,'StartTime',struct('Selected',0,'Value',0),'AutoRepeatTime',struct('Selected',0,'Value',0.1),'Timeout',struct('Selected',0,'Value',0.1),'DelayTime',struct('Selected',0,'Value',0.1),'Signal',struct('SgnName','STEERING_ANGLE_CMD','SgnStartBit',0,'SgnLength',16,'SgnType',0,'ModeValue',-1,'DataType',1,'ByteLayout',0,'Factor',0.0004,'Offset',0,'SgnComment',{{''}},'SgnUnit','rad','Min',-13.1072,'Max',13.1068,'SLDataType','SS_DOUBLE'),'MsgIdNumFormat',0,'MsgComment',{{''}}),'Version',1.2,'general',struct('isFromLib',0)),'OFF',[]}},'GroupId',{{struct('Group',{{'RTICAN'}},'No',1,'Behavior',{{'NAMECHANGE'}},'BlockType',{{'SINK'}},'NameChangeFlag',0),'OFF',[]}},'SFcnRTICANMessage',{{struct('MsgType','TX','SFcnPortType','Scalar','MsgName','STEERING_CMD','MsgIdFormat','STD','MsgId',1,'MsgLength',2,'NumSignals',1,'SampleTime',-1,'StartTime',struct('Selected','no','Value',0),'AutoRepeatTime',struct('Selected','no','Value',0.1),'Timeout',struct('Selected','no','Value',0.1),'Signal',struct('SgnName','STEERING_ANGLE_CMD','SgnStartBit',0,'SgnLength',16,'SgnType','standard','ModeValue',-1,'DataType',['signed int'],'ByteLayout',['little endian'],'Factor',0.0004,'Offset',0,'SLDataType','SS_DOUBLE'),'StatusSelected','no','TimeSelected','no','DeltaTimeSelected','no','DelayTimeSelected','yes','DelayTimeTXCommandSelected','no','EncodeSetUnusedBitsToOne','no','EnableMsgLoopback','no','TriggerPort',struct('Selected','no','TriggerType',0),'EnablePortSelected','no','UserCoding',struct('Selected','no','InterfaceFile','UserEncodingFile','FcnName','UserEncodeFcn','InportSelected','no','InportWidth',1,'OutportSelected','no','OutportWidth',1),'TerminationMsg',struct('Selected','no','Byte0','0x00','Byte1','0x00','Byte2','0x00','Byte3','0x00','Byte4','0x00','Byte5','0x00','Byte6','0x00','Byte7','0x00'),'InitialMsg',struct('Selected','no','Byte0','0x00','Byte1','0x00','Byte2','0x00','Byte3','0x00','Byte4','0x00','Byte5','0x00','Byte6','0x00','Byte7','0x00'),'BoardType','DS1','BoardNo',1,'ControllerNo',1),'OFF',[]}},'TLCFileName',{{'rtican_tx_message','OFF',[]}})  RTISFcnParameters=struct('SFcnRTICANMessage','struct','TLCFileName','char')  RTIBlockParaDefault=struct('BoardTypeNo',4302,'BoardNo',1,'ChannelNo',1,'Parameters',struct('DataFileSupport',struct('DataFileSelectedMaster',0,'DataFileSelectedLocal',0,'DataFileName','','DataFileDate','','SelectedFile',['<no file selected>']),'Options',struct('StatusSelected',1,'TimeSelected',1,'DeltaTimeSelected',1,'DelayTimeSelected',1,'DelayTimeTXCommandSelected',0,'EncodeSetUnusedBitsToOne',0,'EnableMsgLoopback',0,'TriggerPort',struct('Selected',0,'TriggerType','rising'),'EnablePortSelected',0,'SignalOnPortnameSelected',1,'UserCoding',struct('Selected',0,'InterfaceFile','UserEncodingFile','FcnName','UserEncodeFcn','InportSelected',0,'InportWidth',1,'OutportSelected',0,'OutportWidth',1),'TerminationMsg',struct('Selected',0,'Byte0_7','0'),'InitialMsg',struct('Selected',0,'Byte0_7','0')),'Message',struct('MsgOnBlocknameSelected',0,'MsgName',['TX Message'],'MsgIdFormat',0,'MsgId',100,'MsgLength',8,'NumSignals',1,'SampleTime',-1,'StartTime',struct('Selected',0,'Value',0),'AutoRepeatTime',struct('Selected',0,'Value',0.1),'Timeout',struct('Selected',0,'Value',0.1),'DelayTime',struct('Selected',0,'Value',0.1),'Signal',struct('SgnName',['TX signal'],'SgnStartBit',0,'SgnLength',8,'SgnType',0,'ModeValue',-1,'DataType',0,'SLDataType','SS_DOUBLE','ByteLayout',0,'Factor',1,'Offset',0,'Min',0,'Max',255,'SgnComment',{{}},'SgnUnit',''),'MsgIdNumFormat',0,'MsgComment',{{''}}),'Version',1.2,'general',struct('isFromLib',1)),'GroupId',struct('Group',{{'RTICAN'}},'No',1,'Behavior',{{'NAMECHANGE'}},'BlockType',{{'SINK'}},'NameChangeFlag',0),'SFcnRTICANMessage',struct('MsgType','TX','MsgName',['TX Message'],'MsgIdFormat','STD','MsgId',100,'MsgLength',2,'NumSignals',1,'SampleTime',-1,'StartTime',struct('Selected','no','Value',0),'AutoRepeatTime',struct('Selected','no','Value',0.1),'Timeout',struct('Selected','no','Value',0.1),'DelayTime',struct('Selected','no','Value',0.1),'Signal',struct('SgnName',['TX signal'],'SgnStartBit',0,'SgnLength',8,'SgnType','standard','ModeValue',-1,'DataType',['unsigned int'],'ByteLayout',['little endian'],'SLDataType','SS_DOUBLE','Factor',1,'Offset',0),'StatusSelected','yes','TimeSelected','yes','DeltaTimeSelected','yes','DelayTimeSelected','yes','EnablePortSelected','no','EnableMsgLoopback','no','DelayTimeTXCommandSelected','no','EncodeSetUnusedBitsToOne','no','UserCoding',struct('Selected','no','InterfaceFile','UserDecodingFile','FcnName','UserDecodeFcn','InportSelected','no','InportWidth',1,'OutportSelected','no','OutportWidth',1),'TerminationMsg',struct('Selected','no','Byte0','0x00','Byte1','0x00','Byte2','0x00','Byte3','0x00','Byte4','0x00','Byte5','0x00','Byte6','0x00','Byte7','0x00'),'InitialMsg',struct('Selected','no','Byte0','0x00','Byte1','0x00','Byte2','0x00','Byte3','0x00','Byte4','0x00','Byte5','0x00','Byte6','0x00','Byte7','0x00'),'TriggerPort',struct('Selected','no','TriggerType','rising'),'BoardType','DS4302','BoardNo',1,'ControllerNo',1,'SFcnPortType','Scalar'),'TLCFileName','rtican_tx_message')
      settings: AttributesFormatString=Group Id: RTICAN1\n  SourceProductName=dSPACE RTI CAN Blockset
  Simulation State : Display  Commented=on
  TORQUE_ACT : rtican/RTICAN Receive (RX)   Reserved1=[]  Reserved2=[]  Reserved3=[]  Reserved4=[]  SfcnMessage=[]  Msg_Struct=[]  BoardTypeNo=[]  BoardNo=[]  ChannelNo=[]  Parameters=[]  DialogFcn=[]  UnitName=[]  Revision=[]  UnitValues=[]  DSProperties=struct('RTI',struct('Version',uint32(5),'BlockType',struct('isSLSource',uint8(1),'isSLSink',uint8(1),'isHWSource',uint8(0),'isHWSink',uint8(0),'isSetup',uint8(0),'isInline',uint8(1),'isNonInline',uint8(0),'isInterrupt',uint8(0),'isChannelwise',uint8(0)),'IOBoardType','RTICAN','UnitType','MESSAGE','Identifier','RX','DialogType','MSVC','BlockSet','RTICAN','SlaveProcessor','CAN'))  RTIBlockInterface=struct('OutputPortsWidth',int32([1 1 1 1]),'OutputPortsActive',[1 1 1 1],'OutputPortsName',{{'TORQUE_FL_ACT','TORQUE_FR_ACT','TORQUE_RL_ACT','TORQUE_RR_ACT'}},'OutputPortsDataType',{{'SS_DOUBLE','SS_DOUBLE','SS_DOUBLE','SS_DOUBLE'}},'OutputPortsLabel',{{'TORQUE_FL_ACT','TORQUE_FR_ACT','TORQUE_RL_ACT','TORQUE_RR_ACT'}},'OutputPortsLabelMode','ON','InputPortsWidth',int32(0),'InputPortsActive',0,'DialogFcn','rtican_message_interface_gui','BlockDisplay',{{'','center'}},'IconTransparency','on','ParameterTunableNames',{{}},'InitLevel',3,'BlockName',struct('Token',{{'TORQUE_ACT'}}),'SampleTime',{{-1}},'TriggerPort',{{'none'}},'EnablePort',{{'none'}})  RTIBlockParameters=struct('BoardTypeNo',{{1,'OFF',[]}},'BoardNo',{{1,'ON',[1 16]}},'ChannelNo',{{1,'ON',[1 2]}},'Parameters',{{struct('DataFileSupport',struct('DataFileSelectedMaster',1,'DataFileSelectedLocal',1,'DataFileName','c:\users\dell\documents\github\rimac-stageb\challenge-resources\can-db\bus.dbc|','DataFileDate',{{{['02-Jun-2018 15:28:47']}}},'SelectedFile','..\..\challenge-resources\can-db\bus.dbc'),'Options',struct('StatusSelected',0,'TimeSelected',0,'DeltaTimeSelected',0,'BytePortSelected',0,'MessageLengthSelected',0,'TriggerPort',struct('Selected',0,'TriggerType',0),'UserCoding',struct('Selected',0,'InterfaceFile','UserDecodingFile','FcnName','UserDecodeFcn','InportSelected',0,'InportWidth',1,'OutportSelected',0,'OutportWidth',1),'EnablePortSelected',0,'SignalOnPortnameSelected',1,'UseRXService',0),'Message',struct('MsgOnBlocknameSelected',1,'MsgName','TORQUE_ACT','MsgIdFormat',0,'MsgId',7,'MsgLength',8,'NumSignals',4,'SampleTime',-1,'Signal',struct('SgnName',{'TORQUE_FL_ACT','TORQUE_FR_ACT','TORQUE_RL_ACT','TORQUE_RR_ACT'},'SgnStartBit',{0,16,32,48},'SgnLength',{16,16,16,16},'SgnType',{0,0,0,0},'ModeValue',{-1,-1,-1,-1},'DataType',{1,1,1,1},'ByteLayout',{0,0,0,0},'Factor',{0.075,0.075,0.075,0.075},'Offset',{0,0,0,0},'SgnComment',{{''},{''},{''},{''}},'SgnUnit',{'Nm','Nm','Nm','Nm'},'Min',{-2457.6,-2457.6,-2457.6,-2457.6},'Max',{2457.525,2457.525,2457.525,2457.525},'SLDataType',{'SS_DOUBLE','SS_DOUBLE','SS_DOUBLE','SS_DOUBLE'}),'MsgIdNumFormat',0,'MsgComment',{{''}}),'Version',1.2,'general',struct('isFromLib',0)),'OFF',[]}},'GroupId',{{struct('Group',{{'RTICAN'}},'No',1,'Behavior',{{'NAMECHANGE'}},'BlockType',{{'SINK'}},'NameChangeFlag',0),'OFF',[]}},'SFcnRTICANMessage',{{struct('MsgType','RX','SFcnPortType','Scalar','MsgName','TORQUE_ACT','MsgIdFormat','STD','MsgId',7,'MsgLength',8,'NumSignals',4,'SampleTime',-1,'Signal',struct('SgnName',{'TORQUE_FL_ACT','TORQUE_FR_ACT','TORQUE_RL_ACT','TORQUE_RR_ACT'},'SgnStartBit',{0,16,32,48},'SgnLength',{16,16,16,16},'SgnType',{'standard','standard','standard','standard'},'ModeValue',{-1,-1,-1,-1},'DataType',{['signed int'],['signed int'],['signed int'],['signed int']},'ByteLayout',{['little endian'],['little endian'],['little endian'],['little endian']},'Factor',{0.075,0.075,0.075,0.075},'Offset',{0,0,0,0},'SLDataType',{'SS_DOUBLE','SS_DOUBLE','SS_DOUBLE','SS_DOUBLE'}),'StatusSelected','no','TimeSelected','no','DeltaTimeSelected','no','BytePortSelected','no','MessageLengthSelected','no','TriggerPort',struct('Selected','no','TriggerType',0),'UserCoding',struct('Selected','no','InterfaceFile','UserDecodingFile','FcnName','UserDecodeFcn','InportSelected','no','InportWidth',1,'OutportSelected','no','OutportWidth',1),'EnablePortSelected','no','UseRXService','no','BoardType','DS1','BoardNo',1,'ControllerNo',1),'OFF',[]}},'TLCFileName',{{'rtican_rx_message','OFF',[]}})  RTISFcnParameters=struct('SFcnRTICANMessage','struct','TLCFileName','char')  RTIBlockParaDefault=struct('BoardTypeNo',4302,'BoardNo',1,'ChannelNo',1,'Parameters',struct('DataFileSupport',struct('DataFileSelectedMaster',0,'DataFileSelectedLocal',0,'DataFileName','','DataFileDate','','SelectedFile',['<no file selected>']),'Options',struct('StatusSelected',1,'TimeSelected',1,'DeltaTimeSelected',1,'BytePortSelected',0,'MessageLengthSelected',0,'TriggerPort',struct('Selected',0,'TriggerType','rising'),'UserCoding',struct('Selected',0,'InterfaceFile','UserDecodingFile','FcnName','UserDecodeFcn','InportSelected',0,'InportWidth',1,'OutportSelected',0,'OutportWidth',1),'EnablePortSelected',0,'SignalOnPortnameSelected',1,'UseRXService',0),'Message',struct('MsgOnBlocknameSelected',0,'MsgName',['RX Message'],'MsgIdFormat',0,'MsgId',100,'MsgLength',8,'NumSignals',1,'SampleTime',-1,'Signal',struct('SgnName',['RX signal'],'SgnStartBit',0,'SgnLength',8,'SgnType',0,'ModeValue',-1,'DataType',0,'SLDataType','SS_DOUBLE','ByteLayout',0,'Factor',1,'Offset',0,'Min',0,'Max',255,'SgnComment',{{}},'SgnUnit',''),'MsgIdNumFormat',0,'MsgComment',{{''}}),'Version',1.2,'general',struct('isFromLib',1)),'GroupId',struct('Group',{{'RTICAN'}},'No',1,'Behavior',{{'NAMECHANGE'}},'BlockType',{{'SINK'}},'NameChangeFlag',0),'SFcnRTICANMessage',struct('MsgType','RX','MsgName',['RX Message'],'MsgIdFormat','STD','MsgId',100,'MsgLength',8,'NumSignals',1,'SampleTime',-1,'Signal',struct('SgnName',['RX signal'],'SgnStartBit',0,'SgnLength',8,'SgnType','standard','ModeValue',-1,'DataType',['unsigned int'],'ByteLayout',['little endian'],'SLDataType','SS_DOUBLE','Factor',1,'Offset',0),'StatusSelected','yes','TimeSelected','yes','DeltaTimeSelected','yes','BytePortSelected','no','MessageLengthSelected','no','EnablePortSelected','no','UserCoding',struct('Selected','no','InterfaceFile','UserDecodingFile','FcnName','UserDecodeFcn','InportSelected','no','InportWidth',1,'OutportSelected','no','OutportWidth',1),'TriggerPort',struct('Selected','no','TriggerType','rising'),'UseRXService','no','BoardType','DS4302','BoardNo',1,'ControllerNo',1,'SFcnPortType','Scalar'),'TLCFileName','rtican_rx_message')
      settings: AttributesFormatString=Group Id: RTICAN1\n  SourceProductName=dSPACE RTI CAN Blockset
  TORQUE_CMD : rtican/RTICAN Transmit (TX)   Reserved1=[]  Reserved2=[]  Reserved3=[]  Reserved4=[]  SfcnMessage=[]  Msg_Struct=[]  BoardTypeNo=[]  BoardNo=[]  ChannelNo=[]  Parameters=[]  DialogFcn=[]  UnitName=[]  Revision=[]  UnitValues=[]  DSProperties=struct('RTI',struct('Version',uint32(5),'BlockType',struct('isSLSource',uint8(1),'isSLSink',uint8(1),'isHWSource',uint8(0),'isHWSink',uint8(0),'isSetup',uint8(0),'isInline',uint8(1),'isNonInline',uint8(0),'isInterrupt',uint8(0),'isChannelwise',uint8(0)),'IOBoardType','RTICAN','UnitType','MESSAGE','Identifier','TX','DialogType','MSVC','BlockSet','RTICAN','SlaveProcessor','CAN'))  RTIBlockInterface=struct('InputPortsWidth',int32([1 1 1 1]),'InputPortsActive',[1 1 1 1],'InputPortsName',{{'TORQUE_FL_CMD','TORQUE_FR_CMD','TORQUE_RL_CMD','TORQUE_RR_CMD'}},'InputPortsDataType',{{'SS_DOUBLE','SS_DOUBLE','SS_DOUBLE','SS_DOUBLE'}},'OutputPortsWidth',int32([1 1 1 1]),'OutputPortsActive',[1 1 1 1],'OutputPortsName',{{['TX status'],['TX time'],['TX delta time'],['TX delay time']}},'DialogFcn','rtican_message_interface_gui','BlockDisplay',{{'','center'}},'IconTransparency','on','InitLevel',3,'BlockName',struct('Token',{{'TORQUE_CMD'}}),'SampleTime',{{-1}},'TriggerPort',{{'none'}},'EnablePort',{{'none'}})  RTIBlockParameters=struct('BoardTypeNo',{{1,'OFF',[]}},'BoardNo',{{1,'ON',[1 16]}},'ChannelNo',{{1,'ON',[1 2]}},'Parameters',{{struct('DataFileSupport',struct('DataFileSelectedMaster',1,'DataFileSelectedLocal',1,'DataFileName','c:\users\dell\documents\github\rimac-stageb\challenge-resources\can-db\bus.dbc|','DataFileDate',{{{['02-Jun-2018 15:28:47']}}},'SelectedFile','..\..\challenge-resources\can-db\bus.dbc'),'Options',struct('StatusSelected',1,'TimeSelected',1,'DeltaTimeSelected',1,'DelayTimeSelected',1,'DelayTimeTXCommandSelected',0,'EncodeSetUnusedBitsToOne',0,'EnableMsgLoopback',0,'TriggerPort',struct('Selected',0,'TriggerType',0),'EnablePortSelected',0,'SignalOnPortnameSelected',1,'UserCoding',struct('Selected',0,'InterfaceFile','UserEncodingFile','FcnName','UserEncodeFcn','InportSelected',0,'InportWidth',1,'OutportSelected',0,'OutportWidth',1),'TerminationMsg',struct('Selected',0,'Byte0_7','0'),'InitialMsg',struct('Selected',0,'Byte0_7','0')),'Message',struct('MsgOnBlocknameSelected',1,'MsgName','TORQUE_CMD','MsgIdFormat',0,'MsgId',0,'MsgLength',8,'NumSignals',4,'SampleTime',-1,'StartTime',struct('Selected',0,'Value',0),'AutoRepeatTime',struct('Selected',0,'Value',0.1),'Timeout',struct('Selected',0,'Value',0.1),'DelayTime',struct('Selected',0,'Value',0.1),'Signal',struct('SgnName',{'TORQUE_FL_CMD','TORQUE_FR_CMD','TORQUE_RL_CMD','TORQUE_RR_CMD'},'SgnStartBit',{0,16,32,48},'SgnLength',{16,16,16,16},'SgnType',{0,0,0,0},'ModeValue',{-1,-1,-1,-1},'DataType',{1,1,1,1},'ByteLayout',{0,0,0,0},'Factor',{0.075,0.075,0.075,0.075},'Offset',{0,0,0,0},'SgnComment',{{''},{''},{''},{''}},'SgnUnit',{'Nm','Nm','Nm','Nm'},'Min',{-2457.6,-2457.6,-2457.6,-2457.6},'Max',{2457.525,2457.525,2457.525,2457.525},'SLDataType',{'SS_DOUBLE','SS_DOUBLE','SS_DOUBLE','SS_DOUBLE'}),'MsgIdNumFormat',0,'MsgComment',{{''}}),'Version',1.2,'general',struct('isFromLib',0)),'OFF',[]}},'GroupId',{{struct('Group',{{'RTICAN'}},'No',1,'Behavior',{{'NAMECHANGE'}},'BlockType',{{'SINK'}},'NameChangeFlag',0),'OFF',[]}},'SFcnRTICANMessage',{{struct('MsgType','TX','SFcnPortType','Scalar','MsgName','TORQUE_CMD','MsgIdFormat','STD','MsgId',0,'MsgLength',8,'NumSignals',4,'SampleTime',-1,'StartTime',struct('Selected','no','Value',0),'AutoRepeatTime',struct('Selected','no','Value',0.1),'Timeout',struct('Selected','no','Value',0.1),'Signal',struct('SgnName',{'TORQUE_FL_CMD','TORQUE_FR_CMD','TORQUE_RL_CMD','TORQUE_RR_CMD'},'SgnStartBit',{0,16,32,48},'SgnLength',{16,16,16,16},'SgnType',{'standard','standard','standard','standard'},'ModeValue',{-1,-1,-1,-1},'DataType',{['signed int'],['signed int'],['signed int'],['signed int']},'ByteLayout',{['little endian'],['little endian'],['little endian'],['little endian']},'Factor',{0.075,0.075,0.075,0.075},'Offset',{0,0,0,0},'SLDataType',{'SS_DOUBLE','SS_DOUBLE','SS_DOUBLE','SS_DOUBLE'}),'StatusSelected','yes','TimeSelected','yes','DeltaTimeSelected','yes','DelayTimeSelected','yes','DelayTimeTXCommandSelected','no','EncodeSetUnusedBitsToOne','no','EnableMsgLoopback','no','TriggerPort',struct('Selected','no','TriggerType',0),'EnablePortSelected','no','UserCoding',struct('Selected','no','InterfaceFile','UserEncodingFile','FcnName','UserEncodeFcn','InportSelected','no','InportWidth',1,'OutportSelected','no','OutportWidth',1),'TerminationMsg',struct('Selected','no','Byte0','0x00','Byte1','0x00','Byte2','0x00','Byte3','0x00','Byte4','0x00','Byte5','0x00','Byte6','0x00','Byte7','0x00'),'InitialMsg',struct('Selected','no','Byte0','0x00','Byte1','0x00','Byte2','0x00','Byte3','0x00','Byte4','0x00','Byte5','0x00','Byte6','0x00','Byte7','0x00'),'BoardType','DS1','BoardNo',1,'ControllerNo',1),'OFF',[]}},'TLCFileName',{{'rtican_tx_message','OFF',[]}})  RTISFcnParameters=struct('SFcnRTICANMessage','struct','TLCFileName','char')  RTIBlockParaDefault=struct('BoardTypeNo',4302,'BoardNo',1,'ChannelNo',1,'Parameters',struct('DataFileSupport',struct('DataFileSelectedMaster',0,'DataFileSelectedLocal',0,'DataFileName','','DataFileDate','','SelectedFile',['<no file selected>']),'Options',struct('StatusSelected',1,'TimeSelected',1,'DeltaTimeSelected',1,'DelayTimeSelected',1,'DelayTimeTXCommandSelected',0,'EncodeSetUnusedBitsToOne',0,'EnableMsgLoopback',0,'TriggerPort',struct('Selected',0,'TriggerType','rising'),'EnablePortSelected',0,'SignalOnPortnameSelected',1,'UserCoding',struct('Selected',0,'InterfaceFile','UserEncodingFile','FcnName','UserEncodeFcn','InportSelected',0,'InportWidth',1,'OutportSelected',0,'OutportWidth',1),'TerminationMsg',struct('Selected',0,'Byte0_7','0'),'InitialMsg',struct('Selected',0,'Byte0_7','0')),'Message',struct('MsgOnBlocknameSelected',0,'MsgName',['TX Message'],'MsgIdFormat',0,'MsgId',100,'MsgLength',8,'NumSignals',1,'SampleTime',-1,'StartTime',struct('Selected',0,'Value',0),'AutoRepeatTime',struct('Selected',0,'Value',0.1),'Timeout',struct('Selected',0,'Value',0.1),'DelayTime',struct('Selected',0,'Value',0.1),'Signal',struct('SgnName',['TX signal'],'SgnStartBit',0,'SgnLength',8,'SgnType',0,'ModeValue',-1,'DataType',0,'SLDataType','SS_DOUBLE','ByteLayout',0,'Factor',1,'Offset',0,'Min',0,'Max',255,'SgnComment',{{}},'SgnUnit',''),'MsgIdNumFormat',0,'MsgComment',{{''}}),'Version',1.2,'general',struct('isFromLib',1)),'GroupId',struct('Group',{{'RTICAN'}},'No',1,'Behavior',{{'NAMECHANGE'}},'BlockType',{{'SINK'}},'NameChangeFlag',0),'SFcnRTICANMessage',struct('MsgType','TX','MsgName',['TX Message'],'MsgIdFormat','STD','MsgId',100,'MsgLength',2,'NumSignals',1,'SampleTime',-1,'StartTime',struct('Selected','no','Value',0),'AutoRepeatTime',struct('Selected','no','Value',0.1),'Timeout',struct('Selected','no','Value',0.1),'DelayTime',struct('Selected','no','Value',0.1),'Signal',struct('SgnName',['TX signal'],'SgnStartBit',0,'SgnLength',8,'SgnType','standard','ModeValue',-1,'DataType',['unsigned int'],'ByteLayout',['little endian'],'SLDataType','SS_DOUBLE','Factor',1,'Offset',0),'StatusSelected','yes','TimeSelected','yes','DeltaTimeSelected','yes','DelayTimeSelected','yes','EnablePortSelected','no','EnableMsgLoopback','no','DelayTimeTXCommandSelected','no','EncodeSetUnusedBitsToOne','no','UserCoding',struct('Selected','no','InterfaceFile','UserDecodingFile','FcnName','UserDecodeFcn','InportSelected','no','InportWidth',1,'OutportSelected','no','OutportWidth',1),'TerminationMsg',struct('Selected','no','Byte0','0x00','Byte1','0x00','Byte2','0x00','Byte3','0x00','Byte4','0x00','Byte5','0x00','Byte6','0x00','Byte7','0x00'),'InitialMsg',struct('Selected','no','Byte0','0x00','Byte1','0x00','Byte2','0x00','Byte3','0x00','Byte4','0x00','Byte5','0x00','Byte6','0x00','Byte7','0x00'),'TriggerPort',struct('Selected','no','TriggerType','rising'),'BoardType','DS4302','BoardNo',1,'ControllerNo',1,'SFcnPortType','Scalar'),'TLCFileName','rtican_tx_message')
      settings: AttributesFormatString=Group Id: RTICAN1\n  SourceProductName=dSPACE RTI CAN Blockset
  VEL : rtican/RTICAN Receive (RX)   Reserved1=[]  Reserved2=[]  Reserved3=[]  Reserved4=[]  SfcnMessage=[]  Msg_Struct=[]  BoardTypeNo=[]  BoardNo=[]  ChannelNo=[]  Parameters=[]  DialogFcn=[]  UnitName=[]  Revision=[]  UnitValues=[]  DSProperties=struct('RTI',struct('Version',uint32(5),'BlockType',struct('isSLSource',uint8(1),'isSLSink',uint8(1),'isHWSource',uint8(0),'isHWSink',uint8(0),'isSetup',uint8(0),'isInline',uint8(1),'isNonInline',uint8(0),'isInterrupt',uint8(0),'isChannelwise',uint8(0)),'IOBoardType','RTICAN','UnitType','MESSAGE','Identifier','RX','DialogType','MSVC','BlockSet','RTICAN','SlaveProcessor','CAN'))  RTIBlockInterface=struct('OutputPortsWidth',int32([1 1 1 1]),'OutputPortsActive',[1 1 1 1],'OutputPortsName',{{'VEL_X','VEL_Y','VEL_Z','POS_X'}},'OutputPortsDataType',{{'SS_DOUBLE','SS_DOUBLE','SS_DOUBLE','SS_DOUBLE'}},'OutputPortsLabel',{{'VEL_X','VEL_Y','VEL_Z','POS_X'}},'OutputPortsLabelMode','ON','InputPortsWidth',int32(0),'InputPortsActive',0,'DialogFcn','rtican_message_interface_gui','BlockDisplay',{{'','center'}},'IconTransparency','on','ParameterTunableNames',{{}},'InitLevel',3,'BlockName',struct('Token',{{'VEL'}}),'SampleTime',{{-1}},'TriggerPort',{{'none'}},'EnablePort',{{'none'}})  RTIBlockParameters=struct('BoardTypeNo',{{1,'OFF',[]}},'BoardNo',{{1,'ON',[1 16]}},'ChannelNo',{{1,'ON',[1 2]}},'Parameters',{{struct('DataFileSupport',struct('DataFileSelectedMaster',1,'DataFileSelectedLocal',1,'DataFileName','c:\users\dell\documents\github\rimac-stageb\challenge-resources\can-db\bus.dbc|','DataFileDate',{{{['02-Jun-2018 15:28:47']}}},'SelectedFile','..\..\challenge-resources\can-db\bus.dbc'),'Options',struct('StatusSelected',0,'TimeSelected',0,'DeltaTimeSelected',0,'BytePortSelected',0,'MessageLengthSelected',0,'TriggerPort',struct('Selected',0,'TriggerType',0),'UserCoding',struct('Selected',0,'InterfaceFile','UserDecodingFile','FcnName','UserDecodeFcn','InportSelected',0,'InportWidth',1,'OutportSelected',0,'OutportWidth',1),'EnablePortSelected',0,'SignalOnPortnameSelected',1,'UseRXService',0),'Message',struct('MsgOnBlocknameSelected',1,'MsgName','VEL','MsgIdFormat',0,'MsgId',3,'MsgLength',8,'NumSignals',4,'SampleTime',-1,'Signal',struct('SgnName',{'VEL_X','VEL_Y','VEL_Z','POS_X'},'SgnStartBit',{0,16,32,48},'SgnLength',{16,16,16,16},'SgnType',{0,0,0,0},'ModeValue',{-1,-1,-1,-1},'DataType',{1,1,1,1},'ByteLayout',{0,0,0,0},'Factor',{0.002,0.002,0.002,0.005},'Offset',{0,0,0,0},'SgnComment',{{''},{''},{''},{''}},'SgnUnit',{'m/s','m/s','m/s','m'},'Min',{-65.536,-65.536,-65.536,-163.84},'Max',{65.534,65.534,65.534,163.835},'SLDataType',{'SS_DOUBLE','SS_DOUBLE','SS_DOUBLE','SS_DOUBLE'}),'MsgIdNumFormat',0,'MsgComment',{{''}}),'Version',1.2,'general',struct('isFromLib',0)),'OFF',[]}},'GroupId',{{struct('Group',{{'RTICAN'}},'No',1,'Behavior',{{'NAMECHANGE'}},'BlockType',{{'SINK'}},'NameChangeFlag',0),'OFF',[]}},'SFcnRTICANMessage',{{struct('MsgType','RX','SFcnPortType','Scalar','MsgName','VEL','MsgIdFormat','STD','MsgId',3,'MsgLength',8,'NumSignals',4,'SampleTime',-1,'Signal',struct('SgnName',{'VEL_X','VEL_Y','VEL_Z','POS_X'},'SgnStartBit',{0,16,32,48},'SgnLength',{16,16,16,16},'SgnType',{'standard','standard','standard','standard'},'ModeValue',{-1,-1,-1,-1},'DataType',{['signed int'],['signed int'],['signed int'],['signed int']},'ByteLayout',{['little endian'],['little endian'],['little endian'],['little endian']},'Factor',{0.002,0.002,0.002,0.005},'Offset',{0,0,0,0},'SLDataType',{'SS_DOUBLE','SS_DOUBLE','SS_DOUBLE','SS_DOUBLE'}),'StatusSelected','no','TimeSelected','no','DeltaTimeSelected','no','BytePortSelected','no','MessageLengthSelected','no','TriggerPort',struct('Selected','no','TriggerType',0),'UserCoding',struct('Selected','no','InterfaceFile','UserDecodingFile','FcnName','UserDecodeFcn','InportSelected','no','InportWidth',1,'OutportSelected','no','OutportWidth',1),'EnablePortSelected','no','UseRXService','no','BoardType','DS1','BoardNo',1,'ControllerNo',1),'OFF',[]}},'TLCFileName',{{'rtican_rx_message','OFF',[]}})  RTISFcnParameters=struct('SFcnRTICANMessage','struct','TLCFileName','char')  RTIBlockParaDefault=struct('BoardTypeNo',4302,'BoardNo',1,'ChannelNo',1,'Parameters',struct('DataFileSupport',struct('DataFileSelectedMaster',0,'DataFileSelectedLocal',0,'DataFileName','','DataFileDate','','SelectedFile',['<no file selected>']),'Options',struct('StatusSelected',1,'TimeSelected',1,'DeltaTimeSelected',1,'BytePortSelected',0,'MessageLengthSelected',0,'TriggerPort',struct('Selected',0,'TriggerType','rising'),'UserCoding',struct('Selected',0,'InterfaceFile','UserDecodingFile','FcnName','UserDecodeFcn','InportSelected',0,'InportWidth',1,'OutportSelected',0,'OutportWidth',1),'EnablePortSelected',0,'SignalOnPortnameSelected',1,'UseRXService',0),'Message',struct('MsgOnBlocknameSelected',0,'MsgName',['RX Message'],'MsgIdFormat',0,'MsgId',100,'MsgLength',8,'NumSignals',1,'SampleTime',-1,'Signal',struct('SgnName',['RX signal'],'SgnStartBit',0,'SgnLength',8,'SgnType',0,'ModeValue',-1,'DataType',0,'SLDataType','SS_DOUBLE','ByteLayout',0,'Factor',1,'Offset',0,'Min',0,'Max',255,'SgnComment',{{}},'SgnUnit',''),'MsgIdNumFormat',0,'MsgComment',{{''}}),'Version',1.2,'general',struct('isFromLib',1)),'GroupId',struct('Group',{{'RTICAN'}},'No',1,'Behavior',{{'NAMECHANGE'}},'BlockType',{{'SINK'}},'NameChangeFlag',0),'SFcnRTICANMessage',struct('MsgType','RX','MsgName',['RX Message'],'MsgIdFormat','STD','MsgId',100,'MsgLength',8,'NumSignals',1,'SampleTime',-1,'Signal',struct('SgnName',['RX signal'],'SgnStartBit',0,'SgnLength',8,'SgnType','standard','ModeValue',-1,'DataType',['unsigned int'],'ByteLayout',['little endian'],'SLDataType','SS_DOUBLE','Factor',1,'Offset',0),'StatusSelected','yes','TimeSelected','yes','DeltaTimeSelected','yes','BytePortSelected','no','MessageLengthSelected','no','EnablePortSelected','no','UserCoding',struct('Selected','no','InterfaceFile','UserDecodingFile','FcnName','UserDecodeFcn','InportSelected','no','InportWidth',1,'OutportSelected','no','OutportWidth',1),'TriggerPort',struct('Selected','no','TriggerType','rising'),'UseRXService','no','BoardType','DS4302','BoardNo',1,'ControllerNo',1,'SFcnPortType','Scalar'),'TLCFileName','rtican_rx_message')
      settings: AttributesFormatString=Group Id: RTICAN1\n  SourceProductName=dSPACE RTI CAN Blockset
  WHEELSPEED : rtican/RTICAN Receive (RX)   Reserved1=[]  Reserved2=[]  Reserved3=[]  Reserved4=[]  SfcnMessage=[]  Msg_Struct=[]  BoardTypeNo=[]  BoardNo=[]  ChannelNo=[]  Parameters=[]  DialogFcn=[]  UnitName=[]  Revision=[]  UnitValues=[]  DSProperties=struct('RTI',struct('Version',uint32(5),'BlockType',struct('isSLSource',uint8(1),'isSLSink',uint8(1),'isHWSource',uint8(0),'isHWSink',uint8(0),'isSetup',uint8(0),'isInline',uint8(1),'isNonInline',uint8(0),'isInterrupt',uint8(0),'isChannelwise',uint8(0)),'IOBoardType','RTICAN','UnitType','MESSAGE','Identifier','RX','DialogType','MSVC','BlockSet','RTICAN','SlaveProcessor','CAN'))  RTIBlockInterface=struct('OutputPortsWidth',int32([1 1 1 1]),'OutputPortsActive',[1 1 1 1],'OutputPortsName',{{'WHEELSPEED_FL','WHEELSPEED_FR','WHEELSPEED_RL','WHEELSPEED_RR'}},'OutputPortsDataType',{{'SS_DOUBLE','SS_DOUBLE','SS_DOUBLE','SS_DOUBLE'}},'OutputPortsLabel',{{'WHEELSPEED_FL','WHEELSPEED_FR','WHEELSPEED_RL','WHEELSPEED_RR'}},'OutputPortsLabelMode','ON','InputPortsWidth',int32(0),'InputPortsActive',0,'DialogFcn','rtican_message_interface_gui','BlockDisplay',{{'','center'}},'IconTransparency','on','ParameterTunableNames',{{}},'InitLevel',3,'BlockName',struct('Token',{{'WHEELSPEED'}}),'SampleTime',{{-1}},'TriggerPort',{{'none'}},'EnablePort',{{'none'}})  RTIBlockParameters=struct('BoardTypeNo',{{1,'OFF',[]}},'BoardNo',{{1,'ON',[1 16]}},'ChannelNo',{{1,'ON',[1 2]}},'Parameters',{{struct('DataFileSupport',struct('DataFileSelectedMaster',1,'DataFileSelectedLocal',1,'DataFileName','c:\users\dell\documents\github\rimac-stageb\challenge-resources\can-db\bus.dbc|','DataFileDate',{{{['02-Jun-2018 15:28:47']}}},'SelectedFile','..\..\challenge-resources\can-db\bus.dbc'),'Options',struct('StatusSelected',0,'TimeSelected',0,'DeltaTimeSelected',0,'BytePortSelected',0,'MessageLengthSelected',0,'TriggerPort',struct('Selected',0,'TriggerType',0),'UserCoding',struct('Selected',0,'InterfaceFile','UserDecodingFile','FcnName','UserDecodeFcn','InportSelected',0,'InportWidth',1,'OutportSelected',0,'OutportWidth',1),'EnablePortSelected',0,'SignalOnPortnameSelected',1,'UseRXService',0),'Message',struct('MsgOnBlocknameSelected',1,'MsgName','WHEELSPEED','MsgIdFormat',0,'MsgId',6,'MsgLength',8,'NumSignals',4,'SampleTime',-1,'Signal',struct('SgnName',{'WHEELSPEED_FL','WHEELSPEED_FR','WHEELSPEED_RL','WHEELSPEED_RR'},'SgnStartBit',{0,16,32,48},'SgnLength',{16,16,16,16},'SgnType',{0,0,0,0},'ModeValue',{-1,-1,-1,-1},'DataType',{1,1,1,1},'ByteLayout',{0,0,0,0},'Factor',{0.006,0.006,0.006,0.006},'Offset',{0,0,0,0},'SgnComment',{{''},{''},{''},{''}},'SgnUnit',{'rad/s','rad/s','rad/s','rad/s'},'Min',{-196.608,-196.608,-196.608,-196.608},'Max',{196.602,196.602,196.602,196.602},'SLDataType',{'SS_DOUBLE','SS_DOUBLE','SS_DOUBLE','SS_DOUBLE'}),'MsgIdNumFormat',0,'MsgComment',{{''}}),'Version',1.2,'general',struct('isFromLib',0)),'OFF',[]}},'GroupId',{{struct('Group',{{'RTICAN'}},'No',1,'Behavior',{{'NAMECHANGE'}},'BlockType',{{'SINK'}},'NameChangeFlag',0),'OFF',[]}},'SFcnRTICANMessage',{{struct('MsgType','RX','SFcnPortType','Scalar','MsgName','WHEELSPEED','MsgIdFormat','STD','MsgId',6,'MsgLength',8,'NumSignals',4,'SampleTime',-1,'Signal',struct('SgnName',{'WHEELSPEED_FL','WHEELSPEED_FR','WHEELSPEED_RL','WHEELSPEED_RR'},'SgnStartBit',{0,16,32,48},'SgnLength',{16,16,16,16},'SgnType',{'standard','standard','standard','standard'},'ModeValue',{-1,-1,-1,-1},'DataType',{['signed int'],['signed int'],['signed int'],['signed int']},'ByteLayout',{['little endian'],['little endian'],['little endian'],['little endian']},'Factor',{0.006,0.006,0.006,0.006},'Offset',{0,0,0,0},'SLDataType',{'SS_DOUBLE','SS_DOUBLE','SS_DOUBLE','SS_DOUBLE'}),'StatusSelected','no','TimeSelected','no','DeltaTimeSelected','no','BytePortSelected','no','MessageLengthSelected','no','TriggerPort',struct('Selected','no','TriggerType',0),'UserCoding',struct('Selected','no','InterfaceFile','UserDecodingFile','FcnName','UserDecodeFcn','InportSelected','no','InportWidth',1,'OutportSelected','no','OutportWidth',1),'EnablePortSelected','no','UseRXService','no','BoardType','DS1','BoardNo',1,'ControllerNo',1),'OFF',[]}},'TLCFileName',{{'rtican_rx_message','OFF',[]}})  RTISFcnParameters=struct('SFcnRTICANMessage','struct','TLCFileName','char')  RTIBlockParaDefault=struct('BoardTypeNo',4302,'BoardNo',1,'ChannelNo',1,'Parameters',struct('DataFileSupport',struct('DataFileSelectedMaster',0,'DataFileSelectedLocal',0,'DataFileName','','DataFileDate','','SelectedFile',['<no file selected>']),'Options',struct('StatusSelected',1,'TimeSelected',1,'DeltaTimeSelected',1,'BytePortSelected',0,'MessageLengthSelected',0,'TriggerPort',struct('Selected',0,'TriggerType','rising'),'UserCoding',struct('Selected',0,'InterfaceFile','UserDecodingFile','FcnName','UserDecodeFcn','InportSelected',0,'InportWidth',1,'OutportSelected',0,'OutportWidth',1),'EnablePortSelected',0,'SignalOnPortnameSelected',1,'UseRXService',0),'Message',struct('MsgOnBlocknameSelected',0,'MsgName',['RX Message'],'MsgIdFormat',0,'MsgId',100,'MsgLength',8,'NumSignals',1,'SampleTime',-1,'Signal',struct('SgnName',['RX signal'],'SgnStartBit',0,'SgnLength',8,'SgnType',0,'ModeValue',-1,'DataType',0,'SLDataType','SS_DOUBLE','ByteLayout',0,'Factor',1,'Offset',0,'Min',0,'Max',255,'SgnComment',{{}},'SgnUnit',''),'MsgIdNumFormat',0,'MsgComment',{{''}}),'Version',1.2,'general',struct('isFromLib',1)),'GroupId',struct('Group',{{'RTICAN'}},'No',1,'Behavior',{{'NAMECHANGE'}},'BlockType',{{'SINK'}},'NameChangeFlag',0),'SFcnRTICANMessage',struct('MsgType','RX','MsgName',['RX Message'],'MsgIdFormat','STD','MsgId',100,'MsgLength',8,'NumSignals',1,'SampleTime',-1,'Signal',struct('SgnName',['RX signal'],'SgnStartBit',0,'SgnLength',8,'SgnType','standard','ModeValue',-1,'DataType',['unsigned int'],'ByteLayout',['little endian'],'SLDataType','SS_DOUBLE','Factor',1,'Offset',0),'StatusSelected','yes','TimeSelected','yes','DeltaTimeSelected','yes','BytePortSelected','no','MessageLengthSelected','no','EnablePortSelected','no','UserCoding',struct('Selected','no','InterfaceFile','UserDecodingFile','FcnName','UserDecodeFcn','InportSelected','no','InportWidth',1,'OutportSelected','no','OutportWidth',1),'TriggerPort',struct('Selected','no','TriggerType','rising'),'UseRXService','no','BoardType','DS4302','BoardNo',1,'ControllerNo',1,'SFcnPortType','Scalar'),'TLCFileName','rtican_rx_message')
      settings: AttributesFormatString=Group Id: RTICAN1\n  SourceProductName=dSPACE RTI CAN Blockset
  wires:
  Control Algorithm/1(steer) -> [steer]
  Control Algorithm/2(Torque_1) -> [T1]
  Control Algorithm/3(Torque_2) -> [T2]
  Control Algorithm/4(Torque_3) -> [T3]
  Control Algorithm/5(Torque_4) -> [T4]
  FMU/1 -> Bus Creator/1  "pos"
  FMU/6 -> Bus Creator/6  "wheelTorque_act"
  FMU/8 -> Bus Creator/8  "function_Reward"
  FMU/3 -> Bus Creator/3  "acc"
  FMU/5 -> Bus Creator/5  "wheelSpeed"
  FMU/7 -> Bus Creator/7  "offset_Lateral"
  FMU/2 -> Bus Creator/2  "vel"
  FMU/4 -> Bus Creator/4  "angularRate"
  FMU/9 -> Bus Creator/9  "simulation_State"
  Bus Creator/1 -> Bus Selector/1
  Bus Selector/1 -> Reward Function/1  "<function_Reward>"
  Bus Selector/2 -> Simulation State/1  "<simulation_State>"
  [steer] -> STEERING_CMD/1
  [T3] -> TORQUE_CMD/3
  [T4] -> TORQUE_CMD/4
  [T2] -> TORQUE_CMD/2
  [T1] -> TORQUE_CMD/1
  Bus Creator1/1 -> Control Algorithm/1(Feedback)
  VEL/4 -> Bus Creator2/1  "POS_X"
  Bus Creator2/1 -> Bus Creator1/1  "<pos>"
  ACC/4 -> Bus Creator2/2  "POS_Y"
  ACC/2 -> Bus Creator3/2  "ACC_Y"
  ACC/1 -> Bus Creator3/1  "ACC_X"
  ACC/3 -> Bus Creator3/3  "ACC_Z"
  Bus Creator3/1 -> Bus Creator1/3  "Acc"
  VEL/1 -> Bus Creator4/1  "VEL_X"
  VEL/2 -> Bus Creator4/2  "VEL_Y"
  VEL/3 -> Bus Creator4/3  "VEL_Z"
  Bus Creator4/1 -> Bus Creator1/2  "Vel"
  ANGRATE/2 -> Bus Creator5/2  "ANGRATE_YAW"
  ANGRATE/3 -> Bus Creator5/3  "ANGRATE_ROLL"
  ANGRATE/1 -> Bus Creator5/1  "ANGRATE_PITCH"
  Bus Creator5/1 -> Bus Creator1/4  "ang_Rate"
  SIMSTATE/2 -> Bus Creator1/7  "OFFSET_LATERAL"
  SIMSTATE/1 -> Bus Creator1/8  "FUNCTION_REWARD"
  SIMSTATE/3 -> Bus Creator1/9  "SIMULATION_STATE"
  TORQUE_ACT/1 -> Bus Creator6/1  "TORQUE_FL_ACT"
  TORQUE_ACT/2 -> Bus Creator6/2  "TORQUE_FR_ACT"
  TORQUE_ACT/3 -> Bus Creator6/3  "TORQUE_RL_ACT"
  TORQUE_ACT/4 -> Bus Creator6/4  "TORQUE_RR_ACT"
  Bus Creator6/1 -> Bus Creator1/6
  WHEELSPEED/1 -> Bus Creator7/1  "WHEELSPEED_FL"
  WHEELSPEED/2 -> Bus Creator7/2  "WHEELSPEED_FR"
  WHEELSPEED/3 -> Bus Creator7/3  "WHEELSPEED_RL"
  WHEELSPEED/4 -> Bus Creator7/4  "WHEELSPEED_RR"
  Bus Creator7/1 -> Bus Creator1/5
  TORQUE_CMD/1 -> Display/1
  TORQUE_CMD/2 -> Display1/1
  TORQUE_CMD/3 -> Display2/1
  TORQUE_CMD/4 -> Display3/1
  STEERING_CMD/1 -> Display4/1
  SIMSTATE1/1 -> Display5/1
  IC/1 -> SIMSTATE1/3
  Control Algorithm/6("Sim_State ") -> Bus Selector1/1
  Bus Selector1/3 -> IC/1  "<SIMULATION_STATE>"
  Bus Selector1/1 -> SIMSTATE1/1  "<OFFSET_LATERAL>"
  Bus Selector1/2 -> SIMSTATE1/2  "<FUNCTION_REWARD>"
